simulink model "AUV_ControlsPreliminary"  (R2020b)
(part 12 of 62)

      settings: PortSchema="{\"entries\":[{\"content\":{\"sides\":[{\"content\":{\"connectorIds\":[\"LConn1\"]},\"type\":\"ConnectorPlacement.EquallySpacedRectSide\",\"uuid\":\"a971723f-ea37-4e9b-910b-501b94fb0ba2\"},{\"content\":{\"connectorIds\":[\"RConn1\"],\"side\":\"RIGHT\"},\"type\":\"ConnectorPlacement.EquallySpacedRectSide\",\"uuid\":\"e50175c1-005c-4b0b-bced-b882197eaab2\"},{\"content\":{\"connectorIds\":[\"LConn2\"],\"side\":\"TOP\"},\"type\":\"ConnectorPlacement.EquallySpacedRectSide\",\"uuid\":\"2a04a964-d53e-47ee-8c79-d53dd599bafe\"},{\"content\":{\"connectorIds\":[\"RConn2\"],\"side\":\"BOTTOM\"},\"type\":\"ConnectorPlacement.EquallySpacedRectSide\",\"uuid\":\"a0066dd6-a193-491c-afbe-bac00dfc3505\"}]},\"type\":\"ConnectorPlacement.EquallySpacedConnector\",\"uuid\":\"c80211c6-bb24-481b-97ca-2752015f3b18\"}],\"packageUris\":[\"http://schema.mathworks.com/mf0/Connector/19700101\"],\"version\":\"1.0\"}"
  Tile63 : Subsystem  mask(Square Tile){side=side, thickness=thick, color=color1, opacity=opacity}
      mask prompts: side "Side (m) :"; thickness "Thickness (m) :"; color "Color [RGB] :"; opacity "Opacity (0...1) :"
      mask help: This block creates a flat, single, square tile element. The square tile body is mass-less, so it will not have an effect on the dynamic simulation. This square tile element can be used as a graphic reference by itself, or as part of a composite graphic reference made of an array of interconnected tiles. The square tile is aligned with the XY plane, and the block provides frame connector ports to the middle points on each of the four sides of the body of the square - right (+X), left (-X), top (+Y) and bottom (-Y). All dimensions are in meters.
      settings: PortSchema="{\"entries\":[{\"content\":{\"sides\":[{\"content\":{\"connectorIds\":[\"LConn1\"]},\"type\":\"ConnectorPlacement.EquallySpacedRectSide\",\"uuid\":\"a971723f-ea37-4e9b-910b-501b94fb0ba2\"},{\"content\":{\"connectorIds\":[\"RConn1\"],\"side\":\"RIGHT\"},\"type\":\"ConnectorPlacement.EquallySpacedRectSide\",\"uuid\":\"e50175c1-005c-4b0b-bced-b882197eaab2\"},{\"content\":{\"connectorIds\":[\"LConn2\"],\"side\":\"TOP\"},\"type\":\"ConnectorPlacement.EquallySpacedRectSide\",\"uuid\":\"2a04a964-d53e-47ee-8c79-d53dd599bafe\"},{\"content\":{\"connectorIds\":[\"RConn2\"],\"side\":\"BOTTOM\"},\"type\":\"ConnectorPlacement.EquallySpacedRectSide\",\"uuid\":\"a0066dd6-a193-491c-afbe-bac00dfc3505\"}]},\"type\":\"ConnectorPlacement.EquallySpacedConnector\",\"uuid\":\"c80211c6-bb24-481b-97ca-2752015f3b18\"}],\"packageUris\":[\"http://schema.mathworks.com/mf0/Connector/19700101\"],\"version\":\"1.0\"}"
  Tile64 : Subsystem  mask(Square Tile){side=side, thickness=thick, color=color2, opacity=opacity}
      mask prompts: side "Side (m) :"; thickness "Thickness (m) :"; color "Color [RGB] :"; opacity "Opacity (0...1) :"
      mask help: This block creates a flat, single, square tile element. The square tile body is mass-less, so it will not have an effect on the dynamic simulation. This square tile element can be used as a graphic reference by itself, or as part of a composite graphic reference made of an array of interconnected tiles. The square tile is aligned with the XY plane, and the block provides frame connector ports to the middle points on each of the four sides of the body of the square - right (+X), left (-X), top (+Y) and bottom (-Y). All dimensions are in meters.
      settings: PortSchema="{\"entries\":[{\"content\":{\"sides\":[{\"content\":{\"connectorIds\":[\"LConn1\"]},\"type\":\"ConnectorPlacement.EquallySpacedRectSide\",\"uuid\":\"a971723f-ea37-4e9b-910b-501b94fb0ba2\"},{\"content\":{\"connectorIds\":[\"RConn1\"],\"side\":\"RIGHT\"},\"type\":\"ConnectorPlacement.EquallySpacedRectSide\",\"uuid\":\"e50175c1-005c-4b0b-bced-b882197eaab2\"},{\"content\":{\"connectorIds\":[\"LConn2\"],\"side\":\"TOP\"},\"type\":\"ConnectorPlacement.EquallySpacedRectSide\",\"uuid\":\"2a04a964-d53e-47ee-8c79-d53dd599bafe\"},{\"content\":{\"connectorIds\":[\"RConn2\"],\"side\":\"BOTTOM\"},\"type\":\"ConnectorPlacement.EquallySpacedRectSide\",\"uuid\":\"a0066dd6-a193-491c-afbe-bac00dfc3505\"}]},\"type\":\"ConnectorPlacement.EquallySpacedConnector\",\"uuid\":\"c80211c6-bb24-481b-97ca-2752015f3b18\"}],\"packageUris\":[\"http://schema.mathworks.com/mf0/Connector/19700101\"],\"version\":\"1.0\"}"
  Tile65 : Subsystem  mask(Square Tile){side=side, thickness=thick, color=color1, opacity=opacity}
      mask prompts: side "Side (m) :"; thickness "Thickness (m) :"; color "Color [RGB] :"; opacity "Opacity (0...1) :"
      mask help: This block creates a flat, single, square tile element. The square tile body is mass-less, so it will not have an effect on the dynamic simulation. This square tile element can be used as a graphic reference by itself, or as part of a composite graphic reference made of an array of interconnected tiles. The square tile is aligned with the XY plane, and the block provides frame connector ports to the middle points on each of the four sides of the body of the square - right (+X), left (-X), top (+Y) and bottom (-Y). All dimensions are in meters.
      settings: PortSchema="{\"entries\":[{\"content\":{\"sides\":[{\"content\":{\"connectorIds\":[\"LConn1\"]},\"type\":\"ConnectorPlacement.EquallySpacedRectSide\",\"uuid\":\"a971723f-ea37-4e9b-910b-501b94fb0ba2\"},{\"content\":{\"connectorIds\":[\"RConn1\"],\"side\":\"RIGHT\"},\"type\":\"ConnectorPlacement.EquallySpacedRectSide\",\"uuid\":\"e50175c1-005c-4b0b-bced-b882197eaab2\"},{\"content\":{\"connectorIds\":[\"LConn2\"],\"side\":\"TOP\"},\"type\":\"ConnectorPlacement.EquallySpacedRectSide\",\"uuid\":\"2a04a964-d53e-47ee-8c79-d53dd599bafe\"},{\"content\":{\"connectorIds\":[\"RConn2\"],\"side\":\"BOTTOM\"},\"type\":\"ConnectorPlacement.EquallySpacedRectSide\",\"uuid\":\"a0066dd6-a193-491c-afbe-bac00dfc3505\"}]},\"type\":\"ConnectorPlacement.EquallySpacedConnector\",\"uuid\":\"c80211c6-bb24-481b-97ca-2752015f3b18\"}],\"packageUris\":[\"http://schema.mathworks.com/mf0/Connector/19700101\"],\"version\":\"1.0\"}"
  Tile66 : Subsystem  mask(Square Tile){side=side, thickness=thick, color=color2, opacity=opacity}
      mask prompts: side "Side (m) :"; thickness "Thickness (m) :"; color "Color [RGB] :"; opacity "Opacity (0...1) :"
      mask help: This block creates a flat, single, square tile element. The square tile body is mass-less, so it will not have an effect on the dynamic simulation. This square tile element can be used as a graphic reference by itself, or as part of a composite graphic reference made of an array of interconnected tiles. The square tile is aligned with the XY plane, and the block provides frame connector ports to the middle points on each of the four sides of the body of the square - right (+X), left (-X), top (+Y) and bottom (-Y). All dimensions are in meters.
      settings: PortSchema="{\"entries\":[{\"content\":{\"sides\":[{\"content\":{\"connectorIds\":[\"LConn1\"]},\"type\":\"ConnectorPlacement.EquallySpacedRectSide\",\"uuid\":\"a971723f-ea37-4e9b-910b-501b94fb0ba2\"},{\"content\":{\"connectorIds\":[\"RConn1\"],\"side\":\"RIGHT\"},\"type\":\"ConnectorPlacement.EquallySpacedRectSide\",\"uuid\":\"e50175c1-005c-4b0b-bced-b882197eaab2\"},{\"content\":{\"connectorIds\":[\"LConn2\"],\"side\":\"TOP\"},\"type\":\"ConnectorPlacement.EquallySpacedRectSide\",\"uuid\":\"2a04a964-d53e-47ee-8c79-d53dd599bafe\"},{\"content\":{\"connectorIds\":[\"RConn2\"],\"side\":\"BOTTOM\"},\"type\":\"ConnectorPlacement.EquallySpacedRectSide\",\"uuid\":\"a0066dd6-a193-491c-afbe-bac00dfc3505\"}]},\"type\":\"ConnectorPlacement.EquallySpacedConnector\",\"uuid\":\"c80211c6-bb24-481b-97ca-2752015f3b18\"}],\"packageUris\":[\"http://schema.mathworks.com/mf0/Connector/19700101\"],\"version\":\"1.0\"}"
  Tile67 : Subsystem  mask(Square Tile){side=side, thickness=thick, color=color1, opacity=opacity}
      mask prompts: side "Side (m) :"; thickness "Thickness (m) :"; color "Color [RGB] :"; opacity "Opacity (0...1) :"
      mask help: This block creates a flat, single, square tile element. The square tile body is mass-less, so it will not have an effect on the dynamic simulation. This square tile element can be used as a graphic reference by itself, or as part of a composite graphic reference made of an array of interconnected tiles. The square tile is aligned with the XY plane, and the block provides frame connector ports to the middle points on each of the four sides of the body of the square - right (+X), left (-X), top (+Y) and bottom (-Y). All dimensions are in meters.
      settings: PortSchema="{\"entries\":[{\"content\":{\"sides\":[{\"content\":{\"connectorIds\":[\"LConn1\"]},\"type\":\"ConnectorPlacement.EquallySpacedRectSide\",\"uuid\":\"a971723f-ea37-4e9b-910b-501b94fb0ba2\"},{\"content\":{\"connectorIds\":[\"RConn1\"],\"side\":\"RIGHT\"},\"type\":\"ConnectorPlacement.EquallySpacedRectSide\",\"uuid\":\"e50175c1-005c-4b0b-bced-b882197eaab2\"},{\"content\":{\"connectorIds\":[\"LConn2\"],\"side\":\"TOP\"},\"type\":\"ConnectorPlacement.EquallySpacedRectSide\",\"uuid\":\"2a04a964-d53e-47ee-8c79-d53dd599bafe\"},{\"content\":{\"connectorIds\":[\"RConn2\"],\"side\":\"BOTTOM\"},\"type\":\"ConnectorPlacement.EquallySpacedRectSide\",\"uuid\":\"a0066dd6-a193-491c-afbe-bac00dfc3505\"}]},\"type\":\"ConnectorPlacement.EquallySpacedConnector\",\"uuid\":\"c80211c6-bb24-481b-97ca-2752015f3b18\"}],\"packageUris\":[\"http://schema.mathworks.com/mf0/Connector/19700101\"],\"version\":\"1.0\"}"
  Tile68 : Subsystem  mask(Square Tile){side=side, thickness=thick, color=color2, opacity=opacity}
      mask prompts: side "Side (m) :"; thickness "Thickness (m) :"; color "Color [RGB] :"; opacity "Opacity (0...1) :"
      mask help: This block creates a flat, single, square tile element. The square tile body is mass-less, so it will not have an effect on the dynamic simulation. This square tile element can be used as a graphic reference by itself, or as part of a composite graphic reference made of an array of interconnected tiles. The square tile is aligned with the XY plane, and the block provides frame connector ports to the middle points on each of the four sides of the body of the square - right (+X), left (-X), top (+Y) and bottom (-Y). All dimensions are in meters.
      settings: PortSchema="{\"entries\":[{\"content\":{\"sides\":[{\"content\":{\"connectorIds\":[\"LConn1\"]},\"type\":\"ConnectorPlacement.EquallySpacedRectSide\",\"uuid\":\"a971723f-ea37-4e9b-910b-501b94fb0ba2\"},{\"content\":{\"connectorIds\":[\"RConn1\"],\"side\":\"RIGHT\"},\"type\":\"ConnectorPlacement.EquallySpacedRectSide\",\"uuid\":\"e50175c1-005c-4b0b-bced-b882197eaab2\"},{\"content\":{\"connectorIds\":[\"LConn2\"],\"side\":\"TOP\"},\"type\":\"ConnectorPlacement.EquallySpacedRectSide\",\"uuid\":\"2a04a964-d53e-47ee-8c79-d53dd599bafe\"},{\"content\":{\"connectorIds\":[\"RConn2\"],\"side\":\"BOTTOM\"},\"type\":\"ConnectorPlacement.EquallySpacedRectSide\",\"uuid\":\"a0066dd6-a193-491c-afbe-bac00dfc3505\"}]},\"type\":\"ConnectorPlacement.EquallySpacedConnector\",\"uuid\":\"c80211c6-bb24-481b-97ca-2752015f3b18\"}],\"packageUris\":[\"http://schema.mathworks.com/mf0/Connector/19700101\"],\"version\":\"1.0\"}"
  Tile69 : Subsystem  mask(Square Tile){side=side, thickness=thick, color=color1, opacity=opacity}
      mask prompts: side "Side (m) :"; thickness "Thickness (m) :"; color "Color [RGB] :"; opacity "Opacity (0...1) :"
      mask help: This block creates a flat, single, square tile element. The square tile body is mass-less, so it will not have an effect on the dynamic simulation. This square tile element can be used as a graphic reference by itself, or as part of a composite graphic reference made of an array of interconnected tiles. The square tile is aligned with the XY plane, and the block provides frame connector ports to the middle points on each of the four sides of the body of the square - right (+X), left (-X), top (+Y) and bottom (-Y). All dimensions are in meters.
      settings: PortSchema="{\"entries\":[{\"content\":{\"sides\":[{\"content\":{\"connectorIds\":[\"LConn1\"]},\"type\":\"ConnectorPlacement.EquallySpacedRectSide\",\"uuid\":\"a971723f-ea37-4e9b-910b-501b94fb0ba2\"},{\"content\":{\"connectorIds\":[\"RConn1\"],\"side\":\"RIGHT\"},\"type\":\"ConnectorPlacement.EquallySpacedRectSide\",\"uuid\":\"e50175c1-005c-4b0b-bced-b882197eaab2\"},{\"content\":{\"connectorIds\":[\"LConn2\"],\"side\":\"TOP\"},\"type\":\"ConnectorPlacement.EquallySpacedRectSide\",\"uuid\":\"2a04a964-d53e-47ee-8c79-d53dd599bafe\"},{\"content\":{\"connectorIds\":[\"RConn2\"],\"side\":\"BOTTOM\"},\"type\":\"ConnectorPlacement.EquallySpacedRectSide\",\"uuid\":\"a0066dd6-a193-491c-afbe-bac00dfc3505\"}]},\"type\":\"ConnectorPlacement.EquallySpacedConnector\",\"uuid\":\"c80211c6-bb24-481b-97ca-2752015f3b18\"}],\"packageUris\":[\"http://schema.mathworks.com/mf0/Connector/19700101\"],\"version\":\"1.0\"}"
  Tile7 : Subsystem  mask(Square Tile){side=side, thickness=thick, color=color1, opacity=opacity}
      mask prompts: side "Side (m) :"; thickness "Thickness (m) :"; color "Color [RGB] :"; opacity "Opacity (0...1) :"
      mask help: This block creates a flat, single, square tile element. The square tile body is mass-less, so it will not have an effect on the dynamic simulation. This square tile element can be used as a graphic reference by itself, or as part of a composite graphic reference made of an array of interconnected tiles. The square tile is aligned with the XY plane, and the block provides frame connector ports to the middle points on each of the four sides of the body of the square - right (+X), left (-X), top (+Y) and bottom (-Y). All dimensions are in meters.
      settings: PortSchema="{\"entries\":[{\"content\":{\"sides\":[{\"content\":{\"connectorIds\":[\"LConn1\"]},\"type\":\"ConnectorPlacement.EquallySpacedRectSide\",\"uuid\":\"a971723f-ea37-4e9b-910b-501b94fb0ba2\"},{\"content\":{\"connectorIds\":[\"RConn1\"],\"side\":\"RIGHT\"},\"type\":\"ConnectorPlacement.EquallySpacedRectSide\",\"uuid\":\"e50175c1-005c-4b0b-bced-b882197eaab2\"},{\"content\":{\"connectorIds\":[\"LConn2\"],\"side\":\"TOP\"},\"type\":\"ConnectorPlacement.EquallySpacedRectSide\",\"uuid\":\"2a04a964-d53e-47ee-8c79-d53dd599bafe\"},{\"content\":{\"connectorIds\":[\"RConn2\"],\"side\":\"BOTTOM\"},\"type\":\"ConnectorPlacement.EquallySpacedRectSide\",\"uuid\":\"a0066dd6-a193-491c-afbe-bac00dfc3505\"}]},\"type\":\"ConnectorPlacement.EquallySpacedConnector\",\"uuid\":\"c80211c6-bb24-481b-97ca-2752015f3b18\"}],\"packageUris\":[\"http://schema.mathworks.com/mf0/Connector/19700101\"],\"version\":\"1.0\"}"
  Tile70 : Subsystem  mask(Square Tile){side=side, thickness=thick, color=color1, opacity=opacity}
      mask prompts: side "Side (m) :"; thickness "Thickness (m) :"; color "Color [RGB] :"; opacity "Opacity (0...1) :"
      mask help: This block creates a flat, single, square tile element. The square tile body is mass-less, so it will not have an effect on the dynamic simulation. This square tile element can be used as a graphic reference by itself, or as part of a composite graphic reference made of an array of interconnected tiles. The square tile is aligned with the XY plane, and the block provides frame connector ports to the middle points on each of the four sides of the body of the square - right (+X), left (-X), top (+Y) and bottom (-Y). All dimensions are in meters.
      settings: PortSchema="{\"entries\":[{\"content\":{\"sides\":[{\"content\":{\"connectorIds\":[\"LConn1\"]},\"type\":\"ConnectorPlacement.EquallySpacedRectSide\",\"uuid\":\"a971723f-ea37-4e9b-910b-501b94fb0ba2\"},{\"content\":{\"connectorIds\":[\"RConn1\"],\"side\":\"RIGHT\"},\"type\":\"ConnectorPlacement.EquallySpacedRectSide\",\"uuid\":\"e50175c1-005c-4b0b-bced-b882197eaab2\"},{\"content\":{\"connectorIds\":[\"LConn2\"],\"side\":\"TOP\"},\"type\":\"ConnectorPlacement.EquallySpacedRectSide\",\"uuid\":\"2a04a964-d53e-47ee-8c79-d53dd599bafe\"},{\"content\":{\"connectorIds\":[\"RConn2\"],\"side\":\"BOTTOM\"},\"type\":\"ConnectorPlacement.EquallySpacedRectSide\",\"uuid\":\"a0066dd6-a193-491c-afbe-bac00dfc3505\"}]},\"type\":\"ConnectorPlacement.EquallySpacedConnector\",\"uuid\":\"c80211c6-bb24-481b-97ca-2752015f3b18\"}],\"packageUris\":[\"http://schema.mathworks.com/mf0/Connector/19700101\"],\"version\":\"1.0\"}"
  Tile71 : Subsystem  mask(Square Tile){side=side, thickness=thick, color=color1, opacity=opacity}
      mask prompts: side "Side (m) :"; thickness "Thickness (m) :"; color "Color [RGB] :"; opacity "Opacity (0...1) :"
      mask help: This block creates a flat, single, square tile element. The square tile body is mass-less, so it will not have an effect on the dynamic simulation. This square tile element can be used as a graphic reference by itself, or as part of a composite graphic reference made of an array of interconnected tiles. The square tile is aligned with the XY plane, and the block provides frame connector ports to the middle points on each of the four sides of the body of the square - right (+X), left (-X), top (+Y) and bottom (-Y). All dimensions are in meters.
      settings: PortSchema="{\"entries\":[{\"content\":{\"sides\":[{\"content\":{\"connectorIds\":[\"LConn1\"]},\"type\":\"ConnectorPlacement.EquallySpacedRectSide\",\"uuid\":\"a971723f-ea37-4e9b-910b-501b94fb0ba2\"},{\"content\":{\"connectorIds\":[\"RConn1\"],\"side\":\"RIGHT\"},\"type\":\"ConnectorPlacement.EquallySpacedRectSide\",\"uuid\":\"e50175c1-005c-4b0b-bced-b882197eaab2\"},{\"content\":{\"connectorIds\":[\"LConn2\"],\"side\":\"TOP\"},\"type\":\"ConnectorPlacement.EquallySpacedRectSide\",\"uuid\":\"2a04a964-d53e-47ee-8c79-d53dd599bafe\"},{\"content\":{\"connectorIds\":[\"RConn2\"],\"side\":\"BOTTOM\"},\"type\":\"ConnectorPlacement.EquallySpacedRectSide\",\"uuid\":\"a0066dd6-a193-491c-afbe-bac00dfc3505\"}]},\"type\":\"ConnectorPlacement.EquallySpacedConnector\",\"uuid\":\"c80211c6-bb24-481b-97ca-2752015f3b18\"}],\"packageUris\":[\"http://schema.mathworks.com/mf0/Connector/19700101\"],\"version\":\"1.0\"}"
  Tile72 : Subsystem  mask(Square Tile){side=side, thickness=thick, color=color2, opacity=opacity}
      mask prompts: side "Side (m) :"; thickness "Thickness (m) :"; color "Color [RGB] :"; opacity "Opacity (0...1) :"
      mask help: This block creates a flat, single, square tile element. The square tile body is mass-less, so it will not have an effect on the dynamic simulation. This square tile element can be used as a graphic reference by itself, or as part of a composite graphic reference made of an array of interconnected tiles. The square tile is aligned with the XY plane, and the block provides frame connector ports to the middle points on each of the four sides of the body of the square - right (+X), left (-X), top (+Y) and bottom (-Y). All dimensions are in meters.
      settings: PortSchema="{\"entries\":[{\"content\":{\"sides\":[{\"content\":{\"connectorIds\":[\"LConn1\"]},\"type\":\"ConnectorPlacement.EquallySpacedRectSide\",\"uuid\":\"a971723f-ea37-4e9b-910b-501b94fb0ba2\"},{\"content\":{\"connectorIds\":[\"RConn1\"],\"side\":\"RIGHT\"},\"type\":\"ConnectorPlacement.EquallySpacedRectSide\",\"uuid\":\"e50175c1-005c-4b0b-bced-b882197eaab2\"},{\"content\":{\"connectorIds\":[\"LConn2\"],\"side\":\"TOP\"},\"type\":\"ConnectorPlacement.EquallySpacedRectSide\",\"uuid\":\"2a04a964-d53e-47ee-8c79-d53dd599bafe\"},{\"content\":{\"connectorIds\":[\"RConn2\"],\"side\":\"BOTTOM\"},\"type\":\"ConnectorPlacement.EquallySpacedRectSide\",\"uuid\":\"a0066dd6-a193-491c-afbe-bac00dfc3505\"}]},\"type\":\"ConnectorPlacement.EquallySpacedConnector\",\"uuid\":\"c80211c6-bb24-481b-97ca-2752015f3b18\"}],\"packageUris\":[\"http://schema.mathworks.com/mf0/Connector/19700101\"],\"version\":\"1.0\"}"
  Tile73 : Subsystem  mask(Square Tile){side=side, thickness=thick, color=color2, opacity=opacity}
      mask prompts: side "Side (m) :"; thickness "Thickness (m) :"; color "Color [RGB] :"; opacity "Opacity (0...1) :"
      mask help: This block creates a flat, single, square tile element. The square tile body is mass-less, so it will not have an effect on the dynamic simulation. This square tile element can be used as a graphic reference by itself, or as part of a composite graphic reference made of an array of interconnected tiles. The square tile is aligned with the XY plane, and the block provides frame connector ports to the middle points on each of the four sides of the body of the square - right (+X), left (-X), top (+Y) and bottom (-Y). All dimensions are in meters.
      settings: PortSchema="{\"entries\":[{\"content\":{\"sides\":[{\"content\":{\"connectorIds\":[\"LConn1\"]},\"type\":\"ConnectorPlacement.EquallySpacedRectSide\",\"uuid\":\"a971723f-ea37-4e9b-910b-501b94fb0ba2\"},{\"content\":{\"connectorIds\":[\"RConn1\"],\"side\":\"RIGHT\"},\"type\":\"ConnectorPlacement.EquallySpacedRectSide\",\"uuid\":\"e50175c1-005c-4b0b-bced-b882197eaab2\"},{\"content\":{\"connectorIds\":[\"LConn2\"],\"side\":\"TOP\"},\"type\":\"ConnectorPlacement.EquallySpacedRectSide\",\"uuid\":\"2a04a964-d53e-47ee-8c79-d53dd599bafe\"},{\"content\":{\"connectorIds\":[\"RConn2\"],\"side\":\"BOTTOM\"},\"type\":\"ConnectorPlacement.EquallySpacedRectSide\",\"uuid\":\"a0066dd6-a193-491c-afbe-bac00dfc3505\"}]},\"type\":\"ConnectorPlacement.EquallySpacedConnector\",\"uuid\":\"c80211c6-bb24-481b-97ca-2752015f3b18\"}],\"packageUris\":[\"http://schema.mathworks.com/mf0/Connector/19700101\"],\"version\":\"1.0\"}"
  Tile74 : Subsystem  mask(Square Tile){side=side, thickness=thick, color=color2, opacity=opacity}
      mask prompts: side "Side (m) :"; thickness "Thickness (m) :"; color "Color [RGB] :"; opacity "Opacity (0...1) :"
      mask help: This block creates a flat, single, square tile element. The square tile body is mass-less, so it will not have an effect on the dynamic simulation. This square tile element can be used as a graphic reference by itself, or as part of a composite graphic reference made of an array of interconnected tiles. The square tile is aligned with the XY plane, and the block provides frame connector ports to the middle points on each of the four sides of the body of the square - right (+X), left (-X), top (+Y) and bottom (-Y). All dimensions are in meters.
      settings: PortSchema="{\"entries\":[{\"content\":{\"sides\":[{\"content\":{\"connectorIds\":[\"LConn1\"]},\"type\":\"ConnectorPlacement.EquallySpacedRectSide\",\"uuid\":\"a971723f-ea37-4e9b-910b-501b94fb0ba2\"},{\"content\":{\"connectorIds\":[\"RConn1\"],\"side\":\"RIGHT\"},\"type\":\"ConnectorPlacement.EquallySpacedRectSide\",\"uuid\":\"e50175c1-005c-4b0b-bced-b882197eaab2\"},{\"content\":{\"connectorIds\":[\"LConn2\"],\"side\":\"TOP\"},\"type\":\"ConnectorPlacement.EquallySpacedRectSide\",\"uuid\":\"2a04a964-d53e-47ee-8c79-d53dd599bafe\"},{\"content\":{\"connectorIds\":[\"RConn2\"],\"side\":\"BOTTOM\"},\"type\":\"ConnectorPlacement.EquallySpacedRectSide\",\"uuid\":\"a0066dd6-a193-491c-afbe-bac00dfc3505\"}]},\"type\":\"ConnectorPlacement.EquallySpacedConnector\",\"uuid\":\"c80211c6-bb24-481b-97ca-2752015f3b18\"}],\"packageUris\":[\"http://schema.mathworks.com/mf0/Connector/19700101\"],\"version\":\"1.0\"}"
  Tile75 : Subsystem  mask(Square Tile){side=side, thickness=thick, color=color1, opacity=opacity}
      mask prompts: side "Side (m) :"; thickness "Thickness (m) :"; color "Color [RGB] :"; opacity "Opacity (0...1) :"
      mask help: This block creates a flat, single, square tile element. The square tile body is mass-less, so it will not have an effect on the dynamic simulation. This square tile element can be used as a graphic reference by itself, or as part of a composite graphic reference made of an array of interconnected tiles. The square tile is aligned with the XY plane, and the block provides frame connector ports to the middle points on each of the four sides of the body of the square - right (+X), left (-X), top (+Y) and bottom (-Y). All dimensions are in meters.
      settings: PortSchema="{\"entries\":[{\"content\":{\"sides\":[{\"content\":{\"connectorIds\":[\"LConn1\"]},\"type\":\"ConnectorPlacement.EquallySpacedRectSide\",\"uuid\":\"a971723f-ea37-4e9b-910b-501b94fb0ba2\"},{\"content\":{\"connectorIds\":[\"RConn1\"],\"side\":\"RIGHT\"},\"type\":\"ConnectorPlacement.EquallySpacedRectSide\",\"uuid\":\"e50175c1-005c-4b0b-bced-b882197eaab2\"},{\"content\":{\"connectorIds\":[\"LConn2\"],\"side\":\"TOP\"},\"type\":\"ConnectorPlacement.EquallySpacedRectSide\",\"uuid\":\"2a04a964-d53e-47ee-8c79-d53dd599bafe\"},{\"content\":{\"connectorIds\":[\"RConn2\"],\"side\":\"BOTTOM\"},\"type\":\"ConnectorPlacement.EquallySpacedRectSide\",\"uuid\":\"a0066dd6-a193-491c-afbe-bac00dfc3505\"}]},\"type\":\"ConnectorPlacement.EquallySpacedConnector\",\"uuid\":\"c80211c6-bb24-481b-97ca-2752015f3b18\"}],\"packageUris\":[\"http://schema.mathworks.com/mf0/Connector/19700101\"],\"version\":\"1.0\"}"
  Tile76 : Subsystem  mask(Square Tile){side=side, thickness=thick, color=color2, opacity=opacity}
      mask prompts: side "Side (m) :"; thickness "Thickness (m) :"; color "Color [RGB] :"; opacity "Opacity (0...1) :"
      mask help: This block creates a flat, single, square tile element. The square tile body is mass-less, so it will not have an effect on the dynamic simulation. This square tile element can be used as a graphic reference by itself, or as part of a composite graphic reference made of an array of interconnected tiles. The square tile is aligned with the XY plane, and the block provides frame connector ports to the middle points on each of the four sides of the body of the square - right (+X), left (-X), top (+Y) and bottom (-Y). All dimensions are in meters.
      settings: PortSchema="{\"entries\":[{\"content\":{\"sides\":[{\"content\":{\"connectorIds\":[\"LConn1\"]},\"type\":\"ConnectorPlacement.EquallySpacedRectSide\",\"uuid\":\"a971723f-ea37-4e9b-910b-501b94fb0ba2\"},{\"content\":{\"connectorIds\":[\"RConn1\"],\"side\":\"RIGHT\"},\"type\":\"ConnectorPlacement.EquallySpacedRectSide\",\"uuid\":\"e50175c1-005c-4b0b-bced-b882197eaab2\"},{\"content\":{\"connectorIds\":[\"LConn2\"],\"side\":\"TOP\"},\"type\":\"ConnectorPlacement.EquallySpacedRectSide\",\"uuid\":\"2a04a964-d53e-47ee-8c79-d53dd599bafe\"},{\"content\":{\"connectorIds\":[\"RConn2\"],\"side\":\"BOTTOM\"},\"type\":\"ConnectorPlacement.EquallySpacedRectSide\",\"uuid\":\"a0066dd6-a193-491c-afbe-bac00dfc3505\"}]},\"type\":\"ConnectorPlacement.EquallySpacedConnector\",\"uuid\":\"c80211c6-bb24-481b-97ca-2752015f3b18\"}],\"packageUris\":[\"http://schema.mathworks.com/mf0/Connector/19700101\"],\"version\":\"1.0\"}"
  Tile77 : Subsystem  mask(Square Tile){side=side, thickness=thick, color=color1, opacity=opacity}
      mask prompts: side "Side (m) :"; thickness "Thickness (m) :"; color "Color [RGB] :"; opacity "Opacity (0...1) :"
      mask help: This block creates a flat, single, square tile element. The square tile body is mass-less, so it will not have an effect on the dynamic simulation. This square tile element can be used as a graphic reference by itself, or as part of a composite graphic reference made of an array of interconnected tiles. The square tile is aligned with the XY plane, and the block provides frame connector ports to the middle points on each of the four sides of the body of the square - right (+X), left (-X), top (+Y) and bottom (-Y). All dimensions are in meters.
      settings: PortSchema="{\"entries\":[{\"content\":{\"sides\":[{\"content\":{\"connectorIds\":[\"LConn1\"]},\"type\":\"ConnectorPlacement.EquallySpacedRectSide\",\"uuid\":\"a971723f-ea37-4e9b-910b-501b94fb0ba2\"},{\"content\":{\"connectorIds\":[\"RConn1\"],\"side\":\"RIGHT\"},\"type\":\"ConnectorPlacement.EquallySpacedRectSide\",\"uuid\":\"e50175c1-005c-4b0b-bced-b882197eaab2\"},{\"content\":{\"connectorIds\":[\"LConn2\"],\"side\":\"TOP\"},\"type\":\"ConnectorPlacement.EquallySpacedRectSide\",\"uuid\":\"2a04a964-d53e-47ee-8c79-d53dd599bafe\"},{\"content\":{\"connectorIds\":[\"RConn2\"],\"side\":\"BOTTOM\"},\"type\":\"ConnectorPlacement.EquallySpacedRectSide\",\"uuid\":\"a0066dd6-a193-491c-afbe-bac00dfc3505\"}]},\"type\":\"ConnectorPlacement.EquallySpacedConnector\",\"uuid\":\"c80211c6-bb24-481b-97ca-2752015f3b18\"}],\"packageUris\":[\"http://schema.mathworks.com/mf0/Connector/19700101\"],\"version\":\"1.0\"}"
  Tile78 : Subsystem  mask(Square Tile){side=side, thickness=thick, color=color2, opacity=opacity}
      mask prompts: side "Side (m) :"; thickness "Thickness (m) :"; color "Color [RGB] :"; opacity "Opacity (0...1) :"
      mask help: This block creates a flat, single, square tile element. The square tile body is mass-less, so it will not have an effect on the dynamic simulation. This square tile element can be used as a graphic reference by itself, or as part of a composite graphic reference made of an array of interconnected tiles. The square tile is aligned with the XY plane, and the block provides frame connector ports to the middle points on each of the four sides of the body of the square - right (+X), left (-X), top (+Y) and bottom (-Y). All dimensions are in meters.
      settings: PortSchema="{\"entries\":[{\"content\":{\"sides\":[{\"content\":{\"connectorIds\":[\"LConn1\"]},\"type\":\"ConnectorPlacement.EquallySpacedRectSide\",\"uuid\":\"a971723f-ea37-4e9b-910b-501b94fb0ba2\"},{\"content\":{\"connectorIds\":[\"RConn1\"],\"side\":\"RIGHT\"},\"type\":\"ConnectorPlacement.EquallySpacedRectSide\",\"uuid\":\"e50175c1-005c-4b0b-bced-b882197eaab2\"},{\"content\":{\"connectorIds\":[\"LConn2\"],\"side\":\"TOP\"},\"type\":\"ConnectorPlacement.EquallySpacedRectSide\",\"uuid\":\"2a04a964-d53e-47ee-8c79-d53dd599bafe\"},{\"content\":{\"connectorIds\":[\"RConn2\"],\"side\":\"BOTTOM\"},\"type\":\"ConnectorPlacement.EquallySpacedRectSide\",\"uuid\":\"a0066dd6-a193-491c-afbe-bac00dfc3505\"}]},\"type\":\"ConnectorPlacement.EquallySpacedConnector\",\"uuid\":\"c80211c6-bb24-481b-97ca-2752015f3b18\"}],\"packageUris\":[\"http://schema.mathworks.com/mf0/Connector/19700101\"],\"version\":\"1.0\"}"
  Tile79 : Subsystem  mask(Square Tile){side=side, thickness=thick, color=color1, opacity=opacity}
      mask prompts: side "Side (m) :"; thickness "Thickness (m) :"; color "Color [RGB] :"; opacity "Opacity (0...1) :"
      mask help: This block creates a flat, single, square tile element. The square tile body is mass-less, so it will not have an effect on the dynamic simulation. This square tile element can be used as a graphic reference by itself, or as part of a composite graphic reference made of an array of interconnected tiles. The square tile is aligned with the XY plane, and the block provides frame connector ports to the middle points on each of the four sides of the body of the square - right (+X), left (-X), top (+Y) and bottom (-Y). All dimensions are in meters.
      settings: PortSchema="{\"entries\":[{\"content\":{\"sides\":[{\"content\":{\"connectorIds\":[\"LConn1\"]},\"type\":\"ConnectorPlacement.EquallySpacedRectSide\",\"uuid\":\"a971723f-ea37-4e9b-910b-501b94fb0ba2\"},{\"content\":{\"connectorIds\":[\"RConn1\"],\"side\":\"RIGHT\"},\"type\":\"ConnectorPlacement.EquallySpacedRectSide\",\"uuid\":\"e50175c1-005c-4b0b-bced-b882197eaab2\"},{\"content\":{\"connectorIds\":[\"LConn2\"],\"side\":\"TOP\"},\"type\":\"ConnectorPlacement.EquallySpacedRectSide\",\"uuid\":\"2a04a964-d53e-47ee-8c79-d53dd599bafe\"},{\"content\":{\"connectorIds\":[\"RConn2\"],\"side\":\"BOTTOM\"},\"type\":\"ConnectorPlacement.EquallySpacedRectSide\",\"uuid\":\"a0066dd6-a193-491c-afbe-bac00dfc3505\"}]},\"type\":\"ConnectorPlacement.EquallySpacedConnector\",\"uuid\":\"c80211c6-bb24-481b-97ca-2752015f3b18\"}],\"packageUris\":[\"http://schema.mathworks.com/mf0/Connector/19700101\"],\"version\":\"1.0\"}"
  Tile8 : Subsystem  mask(Square Tile){side=side, thickness=thick, color=color2, opacity=opacity}
      mask prompts: side "Side (m) :"; thickness "Thickness (m) :"; color "Color [RGB] :"; opacity "Opacity (0...1) :"
      mask help: This block creates a flat, single, square tile element. The square tile body is mass-less, so it will not have an effect on the dynamic simulation. This square tile element can be used as a graphic reference by itself, or as part of a composite graphic reference made of an array of interconnected tiles. The square tile is aligned with the XY plane, and the block provides frame connector ports to the middle points on each of the four sides of the body of the square - right (+X), left (-X), top (+Y) and bottom (-Y). All dimensions are in meters.
      settings: PortSchema="{\"entries\":[{\"content\":{\"sides\":[{\"content\":{\"connectorIds\":[\"LConn1\"]},\"type\":\"ConnectorPlacement.EquallySpacedRectSide\",\"uuid\":\"a971723f-ea37-4e9b-910b-501b94fb0ba2\"},{\"content\":{\"connectorIds\":[\"RConn1\"],\"side\":\"RIGHT\"},\"type\":\"ConnectorPlacement.EquallySpacedRectSide\",\"uuid\":\"e50175c1-005c-4b0b-bced-b882197eaab2\"},{\"content\":{\"connectorIds\":[\"LConn2\"],\"side\":\"TOP\"},\"type\":\"ConnectorPlacement.EquallySpacedRectSide\",\"uuid\":\"2a04a964-d53e-47ee-8c79-d53dd599bafe\"},{\"content\":{\"connectorIds\":[\"RConn2\"],\"side\":\"BOTTOM\"},\"type\":\"ConnectorPlacement.EquallySpacedRectSide\",\"uuid\":\"a0066dd6-a193-491c-afbe-bac00dfc3505\"}]},\"type\":\"ConnectorPlacement.EquallySpacedConnector\",\"uuid\":\"c80211c6-bb24-481b-97ca-2752015f3b18\"}],\"packageUris\":[\"http://schema.mathworks.com/mf0/Connector/19700101\"],\"version\":\"1.0\"}"
  Tile80 : Subsystem  mask(Square Tile){side=side, thickness=thick, color=color2, opacity=opacity}
      mask prompts: side "Side (m) :"; thickness "Thickness (m) :"; color "Color [RGB] :"; opacity "Opacity (0...1) :"
      mask help: This block creates a flat, single, square tile element. The square tile body is mass-less, so it will not have an effect on the dynamic simulation. This square tile element can be used as a graphic reference by itself, or as part of a composite graphic reference made of an array of interconnected tiles. The square tile is aligned with the XY plane, and the block provides frame connector ports to the middle points on each of the four sides of the body of the square - right (+X), left (-X), top (+Y) and bottom (-Y). All dimensions are in meters.
      settings: PortSchema="{\"entries\":[{\"content\":{\"sides\":[{\"content\":{\"connectorIds\":[\"LConn1\"]},\"type\":\"ConnectorPlacement.EquallySpacedRectSide\",\"uuid\":\"a971723f-ea37-4e9b-910b-501b94fb0ba2\"},{\"content\":{\"connectorIds\":[\"RConn1\"],\"side\":\"RIGHT\"},\"type\":\"ConnectorPlacement.EquallySpacedRectSide\",\"uuid\":\"e50175c1-005c-4b0b-bced-b882197eaab2\"},{\"content\":{\"connectorIds\":[\"LConn2\"],\"side\":\"TOP\"},\"type\":\"ConnectorPlacement.EquallySpacedRectSide\",\"uuid\":\"2a04a964-d53e-47ee-8c79-d53dd599bafe\"},{\"content\":{\"connectorIds\":[\"RConn2\"],\"side\":\"BOTTOM\"},\"type\":\"ConnectorPlacement.EquallySpacedRectSide\",\"uuid\":\"a0066dd6-a193-491c-afbe-bac00dfc3505\"}]},\"type\":\"ConnectorPlacement.EquallySpacedConnector\",\"uuid\":\"c80211c6-bb24-481b-97ca-2752015f3b18\"}],\"packageUris\":[\"http://schema.mathworks.com/mf0/Connector/19700101\"],\"version\":\"1.0\"}"
  Tile81 : Subsystem  mask(Square Tile){side=side, thickness=thick, color=color1, opacity=opacity}
      mask prompts: side "Side (m) :"; thickness "Thickness (m) :"; color "Color [RGB] :"; opacity "Opacity (0...1) :"
      mask help: This block creates a flat, single, square tile element. The square tile body is mass-less, so it will not have an effect on the dynamic simulation. This square tile element can be used as a graphic reference by itself, or as part of a composite graphic reference made of an array of interconnected tiles. The square tile is aligned with the XY plane, and the block provides frame connector ports to the middle points on each of the four sides of the body of the square - right (+X), left (-X), top (+Y) and bottom (-Y). All dimensions are in meters.
      settings: PortSchema="{\"entries\":[{\"content\":{\"sides\":[{\"content\":{\"connectorIds\":[\"LConn1\"]},\"type\":\"ConnectorPlacement.EquallySpacedRectSide\",\"uuid\":\"a971723f-ea37-4e9b-910b-501b94fb0ba2\"},{\"content\":{\"connectorIds\":[\"RConn1\"],\"side\":\"RIGHT\"},\"type\":\"ConnectorPlacement.EquallySpacedRectSide\",\"uuid\":\"e50175c1-005c-4b0b-bced-b882197eaab2\"},{\"content\":{\"connectorIds\":[\"LConn2\"],\"side\":\"TOP\"},\"type\":\"ConnectorPlacement.EquallySpacedRectSide\",\"uuid\":\"2a04a964-d53e-47ee-8c79-d53dd599bafe\"},{\"content\":{\"connectorIds\":[\"RConn2\"],\"side\":\"BOTTOM\"},\"type\":\"ConnectorPlacement.EquallySpacedRectSide\",\"uuid\":\"a0066dd6-a193-491c-afbe-bac00dfc3505\"}]},\"type\":\"ConnectorPlacement.EquallySpacedConnector\",\"uuid\":\"c80211c6-bb24-481b-97ca-2752015f3b18\"}],\"packageUris\":[\"http://schema.mathworks.com/mf0/Connector/19700101\"],\"version\":\"1.0\"}"
  Tile82 : Subsystem  mask(Square Tile){side=side, thickness=thick, color=color2, opacity=opacity}
      mask prompts: side "Side (m) :"; thickness "Thickness (m) :"; color "Color [RGB] :"; opacity "Opacity (0...1) :"
      mask help: This block creates a flat, single, square tile element. The square tile body is mass-less, so it will not have an effect on the dynamic simulation. This square tile element can be used as a graphic reference by itself, or as part of a composite graphic reference made of an array of interconnected tiles. The square tile is aligned with the XY plane, and the block provides frame connector ports to the middle points on each of the four sides of the body of the square - right (+X), left (-X), top (+Y) and bottom (-Y). All dimensions are in meters.
      settings: PortSchema="{\"entries\":[{\"content\":{\"sides\":[{\"content\":{\"connectorIds\":[\"LConn1\"]},\"type\":\"ConnectorPlacement.EquallySpacedRectSide\",\"uuid\":\"a971723f-ea37-4e9b-910b-501b94fb0ba2\"},{\"content\":{\"connectorIds\":[\"RConn1\"],\"side\":\"RIGHT\"},\"type\":\"ConnectorPlacement.EquallySpacedRectSide\",\"uuid\":\"e50175c1-005c-4b0b-bced-b882197eaab2\"},{\"content\":{\"connectorIds\":[\"LConn2\"],\"side\":\"TOP\"},\"type\":\"ConnectorPlacement.EquallySpacedRectSide\",\"uuid\":\"2a04a964-d53e-47ee-8c79-d53dd599bafe\"},{\"content\":{\"connectorIds\":[\"RConn2\"],\"side\":\"BOTTOM\"},\"type\":\"ConnectorPlacement.EquallySpacedRectSide\",\"uuid\":\"a0066dd6-a193-491c-afbe-bac00dfc3505\"}]},\"type\":\"ConnectorPlacement.EquallySpacedConnector\",\"uuid\":\"c80211c6-bb24-481b-97ca-2752015f3b18\"}],\"packageUris\":[\"http://schema.mathworks.com/mf0/Connector/19700101\"],\"version\":\"1.0\"}"
  Tile83 : Subsystem  mask(Square Tile){side=side, thickness=thick, color=color1, opacity=opacity}
      mask prompts: side "Side (m) :"; thickness "Thickness (m) :"; color "Color [RGB] :"; opacity "Opacity (0...1) :"
      mask help: This block creates a flat, single, square tile element. The square tile body is mass-less, so it will not have an effect on the dynamic simulation. This square tile element can be used as a graphic reference by itself, or as part of a composite graphic reference made of an array of interconnected tiles. The square tile is aligned with the XY plane, and the block provides frame connector ports to the middle points on each of the four sides of the body of the square - right (+X), left (-X), top (+Y) and bottom (-Y). All dimensions are in meters.
      settings: PortSchema="{\"entries\":[{\"content\":{\"sides\":[{\"content\":{\"connectorIds\":[\"LConn1\"]},\"type\":\"ConnectorPlacement.EquallySpacedRectSide\",\"uuid\":\"a971723f-ea37-4e9b-910b-501b94fb0ba2\"},{\"content\":{\"connectorIds\":[\"RConn1\"],\"side\":\"RIGHT\"},\"type\":\"ConnectorPlacement.EquallySpacedRectSide\",\"uuid\":\"e50175c1-005c-4b0b-bced-b882197eaab2\"},{\"content\":{\"connectorIds\":[\"LConn2\"],\"side\":\"TOP\"},\"type\":\"ConnectorPlacement.EquallySpacedRectSide\",\"uuid\":\"2a04a964-d53e-47ee-8c79-d53dd599bafe\"},{\"content\":{\"connectorIds\":[\"RConn2\"],\"side\":\"BOTTOM\"},\"type\":\"ConnectorPlacement.EquallySpacedRectSide\",\"uuid\":\"a0066dd6-a193-491c-afbe-bac00dfc3505\"}]},\"type\":\"ConnectorPlacement.EquallySpacedConnector\",\"uuid\":\"c80211c6-bb24-481b-97ca-2752015f3b18\"}],\"packageUris\":[\"http://schema.mathworks.com/mf0/Connector/19700101\"],\"version\":\"1.0\"}"
  Tile84 : Subsystem  mask(Square Tile){side=side, thickness=thick, color=color1, opacity=opacity}
      mask prompts: side "Side (m) :"; thickness "Thickness (m) :"; color "Color [RGB] :"; opacity "Opacity (0...1) :"
      mask help: This block creates a flat, single, square tile element. The square tile body is mass-less, so it will not have an effect on the dynamic simulation. This square tile element can be used as a graphic reference by itself, or as part of a composite graphic reference made of an array of interconnected tiles. The square tile is aligned with the XY plane, and the block provides frame connector ports to the middle points on each of the four sides of the body of the square - right (+X), left (-X), top (+Y) and bottom (-Y). All dimensions are in meters.
      settings: PortSchema="{\"entries\":[{\"content\":{\"sides\":[{\"content\":{\"connectorIds\":[\"LConn1\"]},\"type\":\"ConnectorPlacement.EquallySpacedRectSide\",\"uuid\":\"a971723f-ea37-4e9b-910b-501b94fb0ba2\"},{\"content\":{\"connectorIds\":[\"RConn1\"],\"side\":\"RIGHT\"},\"type\":\"ConnectorPlacement.EquallySpacedRectSide\",\"uuid\":\"e50175c1-005c-4b0b-bced-b882197eaab2\"},{\"content\":{\"connectorIds\":[\"LConn2\"],\"side\":\"TOP\"},\"type\":\"ConnectorPlacement.EquallySpacedRectSide\",\"uuid\":\"2a04a964-d53e-47ee-8c79-d53dd599bafe\"},{\"content\":{\"connectorIds\":[\"RConn2\"],\"side\":\"BOTTOM\"},\"type\":\"ConnectorPlacement.EquallySpacedRectSide\",\"uuid\":\"a0066dd6-a193-491c-afbe-bac00dfc3505\"}]},\"type\":\"ConnectorPlacement.EquallySpacedConnector\",\"uuid\":\"c80211c6-bb24-481b-97ca-2752015f3b18\"}],\"packageUris\":[\"http://schema.mathworks.com/mf0/Connector/19700101\"],\"version\":\"1.0\"}"
  Tile85 : Subsystem  mask(Square Tile){side=side, thickness=thick, color=color2, opacity=opacity}
      mask prompts: side "Side (m) :"; thickness "Thickness (m) :"; color "Color [RGB] :"; opacity "Opacity (0...1) :"
      mask help: This block creates a flat, single, square tile element. The square tile body is mass-less, so it will not have an effect on the dynamic simulation. This square tile element can be used as a graphic reference by itself, or as part of a composite graphic reference made of an array of interconnected tiles. The square tile is aligned with the XY plane, and the block provides frame connector ports to the middle points on each of the four sides of the body of the square - right (+X), left (-X), top (+Y) and bottom (-Y). All dimensions are in meters.
      settings: PortSchema="{\"entries\":[{\"content\":{\"sides\":[{\"content\":{\"connectorIds\":[\"LConn1\"]},\"type\":\"ConnectorPlacement.EquallySpacedRectSide\",\"uuid\":\"a971723f-ea37-4e9b-910b-501b94fb0ba2\"},{\"content\":{\"connectorIds\":[\"RConn1\"],\"side\":\"RIGHT\"},\"type\":\"ConnectorPlacement.EquallySpacedRectSide\",\"uuid\":\"e50175c1-005c-4b0b-bced-b882197eaab2\"},{\"content\":{\"connectorIds\":[\"LConn2\"],\"side\":\"TOP\"},\"type\":\"ConnectorPlacement.EquallySpacedRectSide\",\"uuid\":\"2a04a964-d53e-47ee-8c79-d53dd599bafe\"},{\"content\":{\"connectorIds\":[\"RConn2\"],\"side\":\"BOTTOM\"},\"type\":\"ConnectorPlacement.EquallySpacedRectSide\",\"uuid\":\"a0066dd6-a193-491c-afbe-bac00dfc3505\"}]},\"type\":\"ConnectorPlacement.EquallySpacedConnector\",\"uuid\":\"c80211c6-bb24-481b-97ca-2752015f3b18\"}],\"packageUris\":[\"http://schema.mathworks.com/mf0/Connector/19700101\"],\"version\":\"1.0\"}"
  Tile86 : Subsystem  mask(Square Tile){side=side, thickness=thick, color=color1, opacity=opacity}
      mask prompts: side "Side (m) :"; thickness "Thickness (m) :"; color "Color [RGB] :"; opacity "Opacity (0...1) :"
      mask help: This block creates a flat, single, square tile element. The square tile body is mass-less, so it will not have an effect on the dynamic simulation. This square tile element can be used as a graphic reference by itself, or as part of a composite graphic reference made of an array of interconnected tiles. The square tile is aligned with the XY plane, and the block provides frame connector ports to the middle points on each of the four sides of the body of the square - right (+X), left (-X), top (+Y) and bottom (-Y). All dimensions are in meters.
      settings: PortSchema="{\"entries\":[{\"content\":{\"sides\":[{\"content\":{\"connectorIds\":[\"LConn1\"]},\"type\":\"ConnectorPlacement.EquallySpacedRectSide\",\"uuid\":\"a971723f-ea37-4e9b-910b-501b94fb0ba2\"},{\"content\":{\"connectorIds\":[\"RConn1\"],\"side\":\"RIGHT\"},\"type\":\"ConnectorPlacement.EquallySpacedRectSide\",\"uuid\":\"e50175c1-005c-4b0b-bced-b882197eaab2\"},{\"content\":{\"connectorIds\":[\"LConn2\"],\"side\":\"TOP\"},\"type\":\"ConnectorPlacement.EquallySpacedRectSide\",\"uuid\":\"2a04a964-d53e-47ee-8c79-d53dd599bafe\"},{\"content\":{\"connectorIds\":[\"RConn2\"],\"side\":\"BOTTOM\"},\"type\":\"ConnectorPlacement.EquallySpacedRectSide\",\"uuid\":\"a0066dd6-a193-491c-afbe-bac00dfc3505\"}]},\"type\":\"ConnectorPlacement.EquallySpacedConnector\",\"uuid\":\"c80211c6-bb24-481b-97ca-2752015f3b18\"}],\"packageUris\":[\"http://schema.mathworks.com/mf0/Connector/19700101\"],\"version\":\"1.0\"}"
  Tile87 : Subsystem  mask(Square Tile){side=side, thickness=thick, color=color2, opacity=opacity}
      mask prompts: side "Side (m) :"; thickness "Thickness (m) :"; color "Color [RGB] :"; opacity "Opacity (0...1) :"
      mask help: This block creates a flat, single, square tile element. The square tile body is mass-less, so it will not have an effect on the dynamic simulation. This square tile element can be used as a graphic reference by itself, or as part of a composite graphic reference made of an array of interconnected tiles. The square tile is aligned with the XY plane, and the block provides frame connector ports to the middle points on each of the four sides of the body of the square - right (+X), left (-X), top (+Y) and bottom (-Y). All dimensions are in meters.
      settings: PortSchema="{\"entries\":[{\"content\":{\"sides\":[{\"content\":{\"connectorIds\":[\"LConn1\"]},\"type\":\"ConnectorPlacement.EquallySpacedRectSide\",\"uuid\":\"a971723f-ea37-4e9b-910b-501b94fb0ba2\"},{\"content\":{\"connectorIds\":[\"RConn1\"],\"side\":\"RIGHT\"},\"type\":\"ConnectorPlacement.EquallySpacedRectSide\",\"uuid\":\"e50175c1-005c-4b0b-bced-b882197eaab2\"},{\"content\":{\"connectorIds\":[\"LConn2\"],\"side\":\"TOP\"},\"type\":\"ConnectorPlacement.EquallySpacedRectSide\",\"uuid\":\"2a04a964-d53e-47ee-8c79-d53dd599bafe\"},{\"content\":{\"connectorIds\":[\"RConn2\"],\"side\":\"BOTTOM\"},\"type\":\"ConnectorPlacement.EquallySpacedRectSide\",\"uuid\":\"a0066dd6-a193-491c-afbe-bac00dfc3505\"}]},\"type\":\"ConnectorPlacement.EquallySpacedConnector\",\"uuid\":\"c80211c6-bb24-481b-97ca-2752015f3b18\"}],\"packageUris\":[\"http://schema.mathworks.com/mf0/Connector/19700101\"],\"version\":\"1.0\"}"
  Tile88 : Subsystem  mask(Square Tile){side=side, thickness=thick, color=color1, opacity=opacity}
      mask prompts: side "Side (m) :"; thickness "Thickness (m) :"; color "Color [RGB] :"; opacity "Opacity (0...1) :"
      mask help: This block creates a flat, single, square tile element. The square tile body is mass-less, so it will not have an effect on the dynamic simulation. This square tile element can be used as a graphic reference by itself, or as part of a composite graphic reference made of an array of interconnected tiles. The square tile is aligned with the XY plane, and the block provides frame connector ports to the middle points on each of the four sides of the body of the square - right (+X), left (-X), top (+Y) and bottom (-Y). All dimensions are in meters.
      settings: PortSchema="{\"entries\":[{\"content\":{\"sides\":[{\"content\":{\"connectorIds\":[\"LConn1\"]},\"type\":\"ConnectorPlacement.EquallySpacedRectSide\",\"uuid\":\"a971723f-ea37-4e9b-910b-501b94fb0ba2\"},{\"content\":{\"connectorIds\":[\"RConn1\"],\"side\":\"RIGHT\"},\"type\":\"ConnectorPlacement.EquallySpacedRectSide\",\"uuid\":\"e50175c1-005c-4b0b-bced-b882197eaab2\"},{\"content\":{\"connectorIds\":[\"LConn2\"],\"side\":\"TOP\"},\"type\":\"ConnectorPlacement.EquallySpacedRectSide\",\"uuid\":\"2a04a964-d53e-47ee-8c79-d53dd599bafe\"},{\"content\":{\"connectorIds\":[\"RConn2\"],\"side\":\"BOTTOM\"},\"type\":\"ConnectorPlacement.EquallySpacedRectSide\",\"uuid\":\"a0066dd6-a193-491c-afbe-bac00dfc3505\"}]},\"type\":\"ConnectorPlacement.EquallySpacedConnector\",\"uuid\":\"c80211c6-bb24-481b-97ca-2752015f3b18\"}],\"packageUris\":[\"http://schema.mathworks.com/mf0/Connector/19700101\"],\"version\":\"1.0\"}"
  Tile89 : Subsystem  mask(Square Tile){side=side, thickness=thick, color=color2, opacity=opacity}
      mask prompts: side "Side (m) :"; thickness "Thickness (m) :"; color "Color [RGB] :"; opacity "Opacity (0...1) :"
      mask help: This block creates a flat, single, square tile element. The square tile body is mass-less, so it will not have an effect on the dynamic simulation. This square tile element can be used as a graphic reference by itself, or as part of a composite graphic reference made of an array of interconnected tiles. The square tile is aligned with the XY plane, and the block provides frame connector ports to the middle points on each of the four sides of the body of the square - right (+X), left (-X), top (+Y) and bottom (-Y). All dimensions are in meters.
      settings: PortSchema="{\"entries\":[{\"content\":{\"sides\":[{\"content\":{\"connectorIds\":[\"LConn1\"]},\"type\":\"ConnectorPlacement.EquallySpacedRectSide\",\"uuid\":\"a971723f-ea37-4e9b-910b-501b94fb0ba2\"},{\"content\":{\"connectorIds\":[\"RConn1\"],\"side\":\"RIGHT\"},\"type\":\"ConnectorPlacement.EquallySpacedRectSide\",\"uuid\":\"e50175c1-005c-4b0b-bced-b882197eaab2\"},{\"content\":{\"connectorIds\":[\"LConn2\"],\"side\":\"TOP\"},\"type\":\"ConnectorPlacement.EquallySpacedRectSide\",\"uuid\":\"2a04a964-d53e-47ee-8c79-d53dd599bafe\"},{\"content\":{\"connectorIds\":[\"RConn2\"],\"side\":\"BOTTOM\"},\"type\":\"ConnectorPlacement.EquallySpacedRectSide\",\"uuid\":\"a0066dd6-a193-491c-afbe-bac00dfc3505\"}]},\"type\":\"ConnectorPlacement.EquallySpacedConnector\",\"uuid\":\"c80211c6-bb24-481b-97ca-2752015f3b18\"}],\"packageUris\":[\"http://schema.mathworks.com/mf0/Connector/19700101\"],\"version\":\"1.0\"}"
  Tile9 : Subsystem  mask(Square Tile){side=side, thickness=thick, color=color1, opacity=opacity}
      mask prompts: side "Side (m) :"; thickness "Thickness (m) :"; color "Color [RGB] :"; opacity "Opacity (0...1) :"
      mask help: This block creates a flat, single, square tile element. The square tile body is mass-less, so it will not have an effect on the dynamic simulation. This square tile element can be used as a graphic reference by itself, or as part of a composite graphic reference made of an array of interconnected tiles. The square tile is aligned with the XY plane, and the block provides frame connector ports to the middle points on each of the four sides of the body of the square - right (+X), left (-X), top (+Y) and bottom (-Y). All dimensions are in meters.
      settings: PortSchema="{\"entries\":[{\"content\":{\"sides\":[{\"content\":{\"connectorIds\":[\"LConn1\"]},\"type\":\"ConnectorPlacement.EquallySpacedRectSide\",\"uuid\":\"a971723f-ea37-4e9b-910b-501b94fb0ba2\"},{\"content\":{\"connectorIds\":[\"RConn1\"],\"side\":\"RIGHT\"},\"type\":\"ConnectorPlacement.EquallySpacedRectSide\",\"uuid\":\"e50175c1-005c-4b0b-bced-b882197eaab2\"},{\"content\":{\"connectorIds\":[\"LConn2\"],\"side\":\"TOP\"},\"type\":\"ConnectorPlacement.EquallySpacedRectSide\",\"uuid\":\"2a04a964-d53e-47ee-8c79-d53dd599bafe\"},{\"content\":{\"connectorIds\":[\"RConn2\"],\"side\":\"BOTTOM\"},\"type\":\"ConnectorPlacement.EquallySpacedRectSide\",\"uuid\":\"a0066dd6-a193-491c-afbe-bac00dfc3505\"}]},\"type\":\"ConnectorPlacement.EquallySpacedConnector\",\"uuid\":\"c80211c6-bb24-481b-97ca-2752015f3b18\"}],\"packageUris\":[\"http://schema.mathworks.com/mf0/Connector/19700101\"],\"version\":\"1.0\"}"
  Tile90 : Subsystem  mask(Square Tile){side=side, thickness=thick, color=color1, opacity=opacity}
      mask prompts: side "Side (m) :"; thickness "Thickness (m) :"; color "Color [RGB] :"; opacity "Opacity (0...1) :"
      mask help: This block creates a flat, single, square tile element. The square tile body is mass-less, so it will not have an effect on the dynamic simulation. This square tile element can be used as a graphic reference by itself, or as part of a composite graphic reference made of an array of interconnected tiles. The square tile is aligned with the XY plane, and the block provides frame connector ports to the middle points on each of the four sides of the body of the square - right (+X), left (-X), top (+Y) and bottom (-Y). All dimensions are in meters.
      settings: PortSchema="{\"entries\":[{\"content\":{\"sides\":[{\"content\":{\"connectorIds\":[\"LConn1\"]},\"type\":\"ConnectorPlacement.EquallySpacedRectSide\",\"uuid\":\"a971723f-ea37-4e9b-910b-501b94fb0ba2\"},{\"content\":{\"connectorIds\":[\"RConn1\"],\"side\":\"RIGHT\"},\"type\":\"ConnectorPlacement.EquallySpacedRectSide\",\"uuid\":\"e50175c1-005c-4b0b-bced-b882197eaab2\"},{\"content\":{\"connectorIds\":[\"LConn2\"],\"side\":\"TOP\"},\"type\":\"ConnectorPlacement.EquallySpacedRectSide\",\"uuid\":\"2a04a964-d53e-47ee-8c79-d53dd599bafe\"},{\"content\":{\"connectorIds\":[\"RConn2\"],\"side\":\"BOTTOM\"},\"type\":\"ConnectorPlacement.EquallySpacedRectSide\",\"uuid\":\"a0066dd6-a193-491c-afbe-bac00dfc3505\"}]},\"type\":\"ConnectorPlacement.EquallySpacedConnector\",\"uuid\":\"c80211c6-bb24-481b-97ca-2752015f3b18\"}],\"packageUris\":[\"http://schema.mathworks.com/mf0/Connector/19700101\"],\"version\":\"1.0\"}"
  Tile91 : Subsystem  mask(Square Tile){side=side, thickness=thick, color=color1, opacity=opacity}
      mask prompts: side "Side (m) :"; thickness "Thickness (m) :"; color "Color [RGB] :"; opacity "Opacity (0...1) :"
      mask help: This block creates a flat, single, square tile element. The square tile body is mass-less, so it will not have an effect on the dynamic simulation. This square tile element can be used as a graphic reference by itself, or as part of a composite graphic reference made of an array of interconnected tiles. The square tile is aligned with the XY plane, and the block provides frame connector ports to the middle points on each of the four sides of the body of the square - right (+X), left (-X), top (+Y) and bottom (-Y). All dimensions are in meters.
      settings: PortSchema="{\"entries\":[{\"content\":{\"sides\":[{\"content\":{\"connectorIds\":[\"LConn1\"]},\"type\":\"ConnectorPlacement.EquallySpacedRectSide\",\"uuid\":\"a971723f-ea37-4e9b-910b-501b94fb0ba2\"},{\"content\":{\"connectorIds\":[\"RConn1\"],\"side\":\"RIGHT\"},\"type\":\"ConnectorPlacement.EquallySpacedRectSide\",\"uuid\":\"e50175c1-005c-4b0b-bced-b882197eaab2\"},{\"content\":{\"connectorIds\":[\"LConn2\"],\"side\":\"TOP\"},\"type\":\"ConnectorPlacement.EquallySpacedRectSide\",\"uuid\":\"2a04a964-d53e-47ee-8c79-d53dd599bafe\"},{\"content\":{\"connectorIds\":[\"RConn2\"],\"side\":\"BOTTOM\"},\"type\":\"ConnectorPlacement.EquallySpacedRectSide\",\"uuid\":\"a0066dd6-a193-491c-afbe-bac00dfc3505\"}]},\"type\":\"ConnectorPlacement.EquallySpacedConnector\",\"uuid\":\"c80211c6-bb24-481b-97ca-2752015f3b18\"}],\"packageUris\":[\"http://schema.mathworks.com/mf0/Connector/19700101\"],\"version\":\"1.0\"}"
  Tile92 : Subsystem  mask(Square Tile){side=side, thickness=thick, color=color2, opacity=opacity}
      mask prompts: side "Side (m) :"; thickness "Thickness (m) :"; color "Color [RGB] :"; opacity "Opacity (0...1) :"
      mask help: This block creates a flat, single, square tile element. The square tile body is mass-less, so it will not have an effect on the dynamic simulation. This square tile element can be used as a graphic reference by itself, or as part of a composite graphic reference made of an array of interconnected tiles. The square tile is aligned with the XY plane, and the block provides frame connector ports to the middle points on each of the four sides of the body of the square - right (+X), left (-X), top (+Y) and bottom (-Y). All dimensions are in meters.
      settings: PortSchema="{\"entries\":[{\"content\":{\"sides\":[{\"content\":{\"connectorIds\":[\"LConn1\"]},\"type\":\"ConnectorPlacement.EquallySpacedRectSide\",\"uuid\":\"a971723f-ea37-4e9b-910b-501b94fb0ba2\"},{\"content\":{\"connectorIds\":[\"RConn1\"],\"side\":\"RIGHT\"},\"type\":\"ConnectorPlacement.EquallySpacedRectSide\",\"uuid\":\"e50175c1-005c-4b0b-bced-b882197eaab2\"},{\"content\":{\"connectorIds\":[\"LConn2\"],\"side\":\"TOP\"},\"type\":\"ConnectorPlacement.EquallySpacedRectSide\",\"uuid\":\"2a04a964-d53e-47ee-8c79-d53dd599bafe\"},{\"content\":{\"connectorIds\":[\"RConn2\"],\"side\":\"BOTTOM\"},\"type\":\"ConnectorPlacement.EquallySpacedRectSide\",\"uuid\":\"a0066dd6-a193-491c-afbe-bac00dfc3505\"}]},\"type\":\"ConnectorPlacement.EquallySpacedConnector\",\"uuid\":\"c80211c6-bb24-481b-97ca-2752015f3b18\"}],\"packageUris\":[\"http://schema.mathworks.com/mf0/Connector/19700101\"],\"version\":\"1.0\"}"
  Tile93 : Subsystem  mask(Square Tile){side=side, thickness=thick, color=color2, opacity=opacity}
      mask prompts: side "Side (m) :"; thickness "Thickness (m) :"; color "Color [RGB] :"; opacity "Opacity (0...1) :"
      mask help: This block creates a flat, single, square tile element. The square tile body is mass-less, so it will not have an effect on the dynamic simulation. This square tile element can be used as a graphic reference by itself, or as part of a composite graphic reference made of an array of interconnected tiles. The square tile is aligned with the XY plane, and the block provides frame connector ports to the middle points on each of the four sides of the body of the square - right (+X), left (-X), top (+Y) and bottom (-Y). All dimensions are in meters.
      settings: PortSchema="{\"entries\":[{\"content\":{\"sides\":[{\"content\":{\"connectorIds\":[\"LConn1\"]},\"type\":\"ConnectorPlacement.EquallySpacedRectSide\",\"uuid\":\"a971723f-ea37-4e9b-910b-501b94fb0ba2\"},{\"content\":{\"connectorIds\":[\"RConn1\"],\"side\":\"RIGHT\"},\"type\":\"ConnectorPlacement.EquallySpacedRectSide\",\"uuid\":\"e50175c1-005c-4b0b-bced-b882197eaab2\"},{\"content\":{\"connectorIds\":[\"LConn2\"],\"side\":\"TOP\"},\"type\":\"ConnectorPlacement.EquallySpacedRectSide\",\"uuid\":\"2a04a964-d53e-47ee-8c79-d53dd599bafe\"},{\"content\":{\"connectorIds\":[\"RConn2\"],\"side\":\"BOTTOM\"},\"type\":\"ConnectorPlacement.EquallySpacedRectSide\",\"uuid\":\"a0066dd6-a193-491c-afbe-bac00dfc3505\"}]},\"type\":\"ConnectorPlacement.EquallySpacedConnector\",\"uuid\":\"c80211c6-bb24-481b-97ca-2752015f3b18\"}],\"packageUris\":[\"http://schema.mathworks.com/mf0/Connector/19700101\"],\"version\":\"1.0\"}"
  Tile94 : Subsystem  mask(Square Tile){side=side, thickness=thick, color=color1, opacity=opacity}
      mask prompts: side "Side (m) :"; thickness "Thickness (m) :"; color "Color [RGB] :"; opacity "Opacity (0...1) :"
      mask help: This block creates a flat, single, square tile element. The square tile body is mass-less, so it will not have an effect on the dynamic simulation. This square tile element can be used as a graphic reference by itself, or as part of a composite graphic reference made of an array of interconnected tiles. The square tile is aligned with the XY plane, and the block provides frame connector ports to the middle points on each of the four sides of the body of the square - right (+X), left (-X), top (+Y) and bottom (-Y). All dimensions are in meters.
      settings: PortSchema="{\"entries\":[{\"content\":{\"sides\":[{\"content\":{\"connectorIds\":[\"LConn1\"]},\"type\":\"ConnectorPlacement.EquallySpacedRectSide\",\"uuid\":\"a971723f-ea37-4e9b-910b-501b94fb0ba2\"},{\"content\":{\"connectorIds\":[\"RConn1\"],\"side\":\"RIGHT\"},\"type\":\"ConnectorPlacement.EquallySpacedRectSide\",\"uuid\":\"e50175c1-005c-4b0b-bced-b882197eaab2\"},{\"content\":{\"connectorIds\":[\"LConn2\"],\"side\":\"TOP\"},\"type\":\"ConnectorPlacement.EquallySpacedRectSide\",\"uuid\":\"2a04a964-d53e-47ee-8c79-d53dd599bafe\"},{\"content\":{\"connectorIds\":[\"RConn2\"],\"side\":\"BOTTOM\"},\"type\":\"ConnectorPlacement.EquallySpacedRectSide\",\"uuid\":\"a0066dd6-a193-491c-afbe-bac00dfc3505\"}]},\"type\":\"ConnectorPlacement.EquallySpacedConnector\",\"uuid\":\"c80211c6-bb24-481b-97ca-2752015f3b18\"}],\"packageUris\":[\"http://schema.mathworks.com/mf0/Connector/19700101\"],\"version\":\"1.0\"}"
  Tile95 : Subsystem  mask(Square Tile){side=side, thickness=thick, color=color2, opacity=opacity}
      mask prompts: side "Side (m) :"; thickness "Thickness (m) :"; color "Color [RGB] :"; opacity "Opacity (0...1) :"
      mask help: This block creates a flat, single, square tile element. The square tile body is mass-less, so it will not have an effect on the dynamic simulation. This square tile element can be used as a graphic reference by itself, or as part of a composite graphic reference made of an array of interconnected tiles. The square tile is aligned with the XY plane, and the block provides frame connector ports to the middle points on each of the four sides of the body of the square - right (+X), left (-X), top (+Y) and bottom (-Y). All dimensions are in meters.
      settings: PortSchema="{\"entries\":[{\"content\":{\"sides\":[{\"content\":{\"connectorIds\":[\"LConn1\"]},\"type\":\"ConnectorPlacement.EquallySpacedRectSide\",\"uuid\":\"a971723f-ea37-4e9b-910b-501b94fb0ba2\"},{\"content\":{\"connectorIds\":[\"RConn1\"],\"side\":\"RIGHT\"},\"type\":\"ConnectorPlacement.EquallySpacedRectSide\",\"uuid\":\"e50175c1-005c-4b0b-bced-b882197eaab2\"},{\"content\":{\"connectorIds\":[\"LConn2\"],\"side\":\"TOP\"},\"type\":\"ConnectorPlacement.EquallySpacedRectSide\",\"uuid\":\"2a04a964-d53e-47ee-8c79-d53dd599bafe\"},{\"content\":{\"connectorIds\":[\"RConn2\"],\"side\":\"BOTTOM\"},\"type\":\"ConnectorPlacement.EquallySpacedRectSide\",\"uuid\":\"a0066dd6-a193-491c-afbe-bac00dfc3505\"}]},\"type\":\"ConnectorPlacement.EquallySpacedConnector\",\"uuid\":\"c80211c6-bb24-481b-97ca-2752015f3b18\"}],\"packageUris\":[\"http://schema.mathworks.com/mf0/Connector/19700101\"],\"version\":\"1.0\"}"
  Tile96 : Subsystem  mask(Square Tile){side=side, thickness=thick, color=color1, opacity=opacity}
      mask prompts: side "Side (m) :"; thickness "Thickness (m) :"; color "Color [RGB] :"; opacity "Opacity (0...1) :"
      mask help: This block creates a flat, single, square tile element. The square tile body is mass-less, so it will not have an effect on the dynamic simulation. This square tile element can be used as a graphic reference by itself, or as part of a composite graphic reference made of an array of interconnected tiles. The square tile is aligned with the XY plane, and the block provides frame connector ports to the middle points on each of the four sides of the body of the square - right (+X), left (-X), top (+Y) and bottom (-Y). All dimensions are in meters.
      settings: PortSchema="{\"entries\":[{\"content\":{\"sides\":[{\"content\":{\"connectorIds\":[\"LConn1\"]},\"type\":\"ConnectorPlacement.EquallySpacedRectSide\",\"uuid\":\"a971723f-ea37-4e9b-910b-501b94fb0ba2\"},{\"content\":{\"connectorIds\":[\"RConn1\"],\"side\":\"RIGHT\"},\"type\":\"ConnectorPlacement.EquallySpacedRectSide\",\"uuid\":\"e50175c1-005c-4b0b-bced-b882197eaab2\"},{\"content\":{\"connectorIds\":[\"LConn2\"],\"side\":\"TOP\"},\"type\":\"ConnectorPlacement.EquallySpacedRectSide\",\"uuid\":\"2a04a964-d53e-47ee-8c79-d53dd599bafe\"},{\"content\":{\"connectorIds\":[\"RConn2\"],\"side\":\"BOTTOM\"},\"type\":\"ConnectorPlacement.EquallySpacedRectSide\",\"uuid\":\"a0066dd6-a193-491c-afbe-bac00dfc3505\"}]},\"type\":\"ConnectorPlacement.EquallySpacedConnector\",\"uuid\":\"c80211c6-bb24-481b-97ca-2752015f3b18\"}],\"packageUris\":[\"http://schema.mathworks.com/mf0/Connector/19700101\"],\"version\":\"1.0\"}"
  Tile97 : Subsystem  mask(Square Tile){side=side, thickness=thick, color=color2, opacity=opacity}
      mask prompts: side "Side (m) :"; thickness "Thickness (m) :"; color "Color [RGB] :"; opacity "Opacity (0...1) :"
      mask help: This block creates a flat, single, square tile element. The square tile body is mass-less, so it will not have an effect on the dynamic simulation. This square tile element can be used as a graphic reference by itself, or as part of a composite graphic reference made of an array of interconnected tiles. The square tile is aligned with the XY plane, and the block provides frame connector ports to the middle points on each of the four sides of the body of the square - right (+X), left (-X), top (+Y) and bottom (-Y). All dimensions are in meters.
      settings: PortSchema="{\"entries\":[{\"content\":{\"sides\":[{\"content\":{\"connectorIds\":[\"LConn1\"]},\"type\":\"ConnectorPlacement.EquallySpacedRectSide\",\"uuid\":\"a971723f-ea37-4e9b-910b-501b94fb0ba2\"},{\"content\":{\"connectorIds\":[\"RConn1\"],\"side\":\"RIGHT\"},\"type\":\"ConnectorPlacement.EquallySpacedRectSide\",\"uuid\":\"e50175c1-005c-4b0b-bced-b882197eaab2\"},{\"content\":{\"connectorIds\":[\"LConn2\"],\"side\":\"TOP\"},\"type\":\"ConnectorPlacement.EquallySpacedRectSide\",\"uuid\":\"2a04a964-d53e-47ee-8c79-d53dd599bafe\"},{\"content\":{\"connectorIds\":[\"RConn2\"],\"side\":\"BOTTOM\"},\"type\":\"ConnectorPlacement.EquallySpacedRectSide\",\"uuid\":\"a0066dd6-a193-491c-afbe-bac00dfc3505\"}]},\"type\":\"ConnectorPlacement.EquallySpacedConnector\",\"uuid\":\"c80211c6-bb24-481b-97ca-2752015f3b18\"}],\"packageUris\":[\"http://schema.mathworks.com/mf0/Connector/19700101\"],\"version\":\"1.0\"}"
  Tile98 : Subsystem  mask(Square Tile){side=side, thickness=thick, color=color1, opacity=opacity}
      mask prompts: side "Side (m) :"; thickness "Thickness (m) :"; color "Color [RGB] :"; opacity "Opacity (0...1) :"
      mask help: This block creates a flat, single, square tile element. The square tile body is mass-less, so it will not have an effect on the dynamic simulation. This square tile element can be used as a graphic reference by itself, or as part of a composite graphic reference made of an array of interconnected tiles. The square tile is aligned with the XY plane, and the block provides frame connector ports to the middle points on each of the four sides of the body of the square - right (+X), left (-X), top (+Y) and bottom (-Y). All dimensions are in meters.
      settings: PortSchema="{\"entries\":[{\"content\":{\"sides\":[{\"content\":{\"connectorIds\":[\"LConn1\"]},\"type\":\"ConnectorPlacement.EquallySpacedRectSide\",\"uuid\":\"a971723f-ea37-4e9b-910b-501b94fb0ba2\"},{\"content\":{\"connectorIds\":[\"RConn1\"],\"side\":\"RIGHT\"},\"type\":\"ConnectorPlacement.EquallySpacedRectSide\",\"uuid\":\"e50175c1-005c-4b0b-bced-b882197eaab2\"},{\"content\":{\"connectorIds\":[\"LConn2\"],\"side\":\"TOP\"},\"type\":\"ConnectorPlacement.EquallySpacedRectSide\",\"uuid\":\"2a04a964-d53e-47ee-8c79-d53dd599bafe\"},{\"content\":{\"connectorIds\":[\"RConn2\"],\"side\":\"BOTTOM\"},\"type\":\"ConnectorPlacement.EquallySpacedRectSide\",\"uuid\":\"a0066dd6-a193-491c-afbe-bac00dfc3505\"}]},\"type\":\"ConnectorPlacement.EquallySpacedConnector\",\"uuid\":\"c80211c6-bb24-481b-97ca-2752015f3b18\"}],\"packageUris\":[\"http://schema.mathworks.com/mf0/Connector/19700101\"],\"version\":\"1.0\"}"
  Tile99 : Subsystem  mask(Square Tile){side=side, thickness=thick, color=color2, opacity=opacity}
      mask prompts: side "Side (m) :"; thickness "Thickness (m) :"; color "Color [RGB] :"; opacity "Opacity (0...1) :"
      mask help: This block creates a flat, single, square tile element. The square tile body is mass-less, so it will not have an effect on the dynamic simulation. This square tile element can be used as a graphic reference by itself, or as part of a composite graphic reference made of an array of interconnected tiles. The square tile is aligned with the XY plane, and the block provides frame connector ports to the middle points on each of the four sides of the body of the square - right (+X), left (-X), top (+Y) and bottom (-Y). All dimensions are in meters.
      settings: PortSchema="{\"entries\":[{\"content\":{\"sides\":[{\"content\":{\"connectorIds\":[\"LConn1\"]},\"type\":\"ConnectorPlacement.EquallySpacedRectSide\",\"uuid\":\"a971723f-ea37-4e9b-910b-501b94fb0ba2\"},{\"content\":{\"connectorIds\":[\"RConn1\"],\"side\":\"RIGHT\"},\"type\":\"ConnectorPlacement.EquallySpacedRectSide\",\"uuid\":\"e50175c1-005c-4b0b-bced-b882197eaab2\"},{\"content\":{\"connectorIds\":[\"LConn2\"],\"side\":\"TOP\"},\"type\":\"ConnectorPlacement.EquallySpacedRectSide\",\"uuid\":\"2a04a964-d53e-47ee-8c79-d53dd599bafe\"},{\"content\":{\"connectorIds\":[\"RConn2\"],\"side\":\"BOTTOM\"},\"type\":\"ConnectorPlacement.EquallySpacedRectSide\",\"uuid\":\"a0066dd6-a193-491c-afbe-bac00dfc3505\"}]},\"type\":\"ConnectorPlacement.EquallySpacedConnector\",\"uuid\":\"c80211c6-bb24-481b-97ca-2752015f3b18\"}],\"packageUris\":[\"http://schema.mathworks.com/mf0/Connector/19700101\"],\"version\":\"1.0\"}"
  F : PMIOPort  Side=Left
  connections:
  F/RConn1 -- Tile1/LConn1
  Tile2/LConn1 -- Tile1/RConn1
  Tile4/LConn1 -- Tile3/RConn1
  Tile2/RConn1 -- Tile3/LConn1
  Tile6/RConn1 -- Tile7/LConn1
  Tile8/LConn1 -- Tile7/RConn1
  Tile6/LConn1 -- Tile5/RConn1
  Tile5/LConn1 -- Tile4/RConn1
  Tile10/LConn1 -- Tile9/RConn1
  Tile9/LConn1 -- Tile8/RConn1
  Tile15/LConn1 -- Tile14/RConn1
  Tile16/LConn1 -- Tile15/RConn1
  Tile16/RConn1 -- Tile17/LConn1
  Tile18/LConn1 -- Tile17/RConn1
  Tile11/LConn1 -- Tile19/RConn1
  Tile19/LConn1 -- Tile18/RConn1
  Tile12/RConn1 -- Tile13/LConn1
  Tile14/LConn1 -- Tile13/RConn1
  Tile12/LConn2 -- Tile1/RConn2
  Tile20/LConn1 -- Tile11/RConn1
  Tile24/LConn2 -- Tile21/RConn2
  Tile26/LConn1 -- Tile25/RConn1
  Tile24/RConn1 -- Tile25/LConn1
  Tile31/LConn1 -- Tile30/RConn1
  Tile30/LConn1 -- Tile29/RConn1
  Tile23/LConn1 -- Tile31/RConn1
  Tile28/RConn1 -- Tile29/LConn1
  Tile28/LConn1 -- Tile27/RConn1
  Tile27/LConn1 -- Tile26/RConn1
  Tile36/LConn1 -- Tile35/RConn1
  Tile37/LConn1 -- Tile36/RConn1
  Tile22/LConn1 -- Tile40/RConn1
  Tile37/RConn1 -- Tile38/LConn1
  Tile40/LConn1 -- Tile39/RConn1
  Tile39/LConn1 -- Tile38/RConn1
  Tile32/RConn1 -- Tile34/LConn1
  Tile35/LConn1 -- Tile34/RConn1
  Tile32/LConn1 -- Tile21/RConn1
  Tile33/LConn1 -- Tile23/RConn1
  Tile21/LConn2 -- Tile12/RConn2
  Tile43/LConn1 -- Tile41/RConn1
  Tile43/RConn1 -- Tile44/LConn1
  Tile49/LConn1 -- Tile48/RConn1
  Tile50/LConn1 -- Tile49/RConn1
  Tile42/LConn1 -- Tile50/RConn1
  Tile47/RConn1 -- Tile48/LConn1
  Tile47/LConn1 -- Tile46/RConn1
  Tile46/LConn1 -- Tile45/RConn1
  Tile45/LConn1 -- Tile44/RConn1
  Tile41/LConn2 -- Tile24/RConn2
  Tile55/LConn1 -- Tile54/RConn1
  Tile56/LConn1 -- Tile55/RConn1
  Tile56/RConn1 -- Tile57/LConn1
  Tile58/LConn1 -- Tile57/RConn1
  Tile52/RConn1 -- Tile53/LConn1
  Tile51/LConn1 -- Tile59/RConn1
  Tile60/LConn1 -- Tile51/RConn1
  Tile54/LConn1 -- Tile53/RConn1
  Tile59/LConn1 -- Tile58/RConn1
  Tile52/LConn2 -- Tile41/RConn2
  Tile109/LConn1 -- Tile108/RConn1
  Tile110/LConn1 -- Tile101/RConn1
  Tile91/LConn2 -- Tile74/RConn2
  Tile95/LConn1 -- Tile94/RConn1
  Tile97/RConn1 -- Tile98/LConn1
  Tile108/LConn1 -- Tile107/RConn1
  Tile100/LConn1 -- Tile99/RConn1
  Tile99/LConn1 -- Tile98/RConn1
  Tile93/RConn1 -- Tile94/LConn1
  Tile85/LConn1 -- Tile84/RConn1
  Tile89/LConn1 -- Tile88/RConn1
  Tile93/LConn1 -- Tile91/RConn1
  Tile90/LConn1 -- Tile89/RConn1
  Tile87/RConn1 -- Tile88/LConn1
  Tile72/LConn1 -- Tile90/RConn1
  Tile96/LConn1 -- Tile95/RConn1
  Tile87/LConn1 -- Tile86/RConn1
  Tile105/LConn1 -- Tile104/RConn1
  Tile86/LConn1 -- Tile85/RConn1
  Tile77/LConn1 -- Tile76/RConn1
  Tile78/LConn1 -- Tile77/RConn1
  Tile82/RConn1 -- Tile84/LConn1
  Tile78/RConn1 -- Tile79/LConn1
  Tile73/LConn1 -- Tile81/RConn1
  Tile80/LConn1 -- Tile79/RConn1
  Tile81/LConn1 -- Tile80/RConn1
  Tile76/LConn1 -- Tile75/RConn1
  Tile74/LConn2 -- Tile71/RConn2
  Tile92/LConn1 -- Tile100/RConn1
  Tile104/LConn1 -- Tile103/RConn1
  Tile102/LConn2 -- Tile91/RConn2
  Tile83/LConn1 -- Tile73/RConn1
  Tile106/RConn1 -- Tile107/LConn1
  Tile74/RConn1 -- Tile75/LConn1
  Tile97/LConn1 -- Tile96/RConn1
  Tile106/LConn1 -- Tile105/RConn1
  Tile101/LConn1 -- Tile109/RConn1
  Tile82/LConn1 -- Tile71/RConn1
  Tile102/RConn1 -- Tile103/LConn1
  Tile1/LConn2 -- Tile102/RConn2
  Tile70/LConn1 -- Tile61/RConn1
  Tile69/LConn1 -- Tile68/RConn1
  Tile62/RConn1 -- Tile63/LConn1
  Tile61/LConn1 -- Tile69/RConn1
  Tile66/RConn1 -- Tile67/LConn1
  Tile68/LConn1 -- Tile67/RConn1
  Tile65/LConn1 -- Tile64/RConn1
  Tile66/LConn1 -- Tile65/RConn1
  Tile64/LConn1 -- Tile63/RConn1
  Tile62/RConn2 -- Tile71/LConn2
  Tile70/RConn1 -- Tile118/LConn1
  Tile72/RConn1 -- Tile121/LConn1
  Tile83/RConn1 -- Tile119/LConn1
  Tile92/RConn1 -- Tile111/LConn1
  Tile110/RConn1 -- Tile112/LConn1
  Tile10/RConn1 -- Tile120/LConn1
  Tile20/RConn1 -- Tile113/LConn1
  Tile22/RConn1 -- Tile115/LConn1
  Tile33/RConn1 -- Tile114/LConn1
  Tile42/RConn1 -- Tile116/LConn1
  Tile60/RConn1 -- Tile117/LConn1
  Tile152/RConn1 -- Tile134/LConn1
  Tile147/RConn1 -- Tile133/LConn1
  Tile141/RConn1 -- Tile132/LConn1
  Tile140/RConn1 -- Tile130/LConn1
  Tile122/RConn1 -- Tile137/LConn1
  Tile144/RConn1 -- Tile131/LConn1
  Tile127/RConn1 -- Tile129/LConn1
  Tile160/RConn1 -- Tile136/LConn1
  Tile156/RConn1 -- Tile138/LConn1
  Tile153/LConn1 -- Tile154/RConn1
  Tile124/LConn1 -- Tile125/RConn1
  Tile160/LConn1 -- Tile157/RConn1
  Tile157/LConn1 -- Tile159/RConn1
  Tile164/LConn1 -- Tile123/RConn1
  Tile156/LConn1 -- Tile163/RConn1
  Tile163/LConn1 -- Tile161/RConn1
  Tile127/LConn1 -- Tile124/RConn1
  Tile155/LConn1 -- Tile153/RConn1
  Tile152/LConn1 -- Tile150/RConn1
  Tile147/LConn1 -- Tile149/RConn1
  Tile141/LConn1 -- Tile146/RConn1
  Tile150/LConn1 -- Tile151/RConn1
  Tile142/LConn1 -- Tile143/RConn1
  Tile146/LConn1 -- Tile145/RConn1
  Tile140/LConn1 -- Tile126/RConn1
  Tile162/LConn1 -- Tile158/RConn1
  Tile126/LConn1 -- Tile139/RConn1
  Tile164/RConn1 -- Tile128/LConn1
  Tile144/LConn1 -- Tile142/RConn1
  Tile123/LConn1 -- Tile165/RConn1
  Tile122/LConn1 -- Tile162/RConn1
  Tile149/LConn1 -- Tile148/RConn1
  Tile155/RConn1 -- Tile135/LConn1
  Tile118/RConn1 -- Tile154/LConn1
  Tile121/RConn1 -- Tile161/LConn1
  Tile119/RConn1 -- Tile159/LConn1
  Tile111/RConn1 -- Tile165/LConn1
  Tile112/RConn1 -- Tile125/LConn1
  Tile120/RConn1 -- Tile158/LConn1
  Tile113/RConn1 -- Tile139/LConn1
  Tile115/RConn1 -- Tile145/LConn1
  Tile114/RConn1 -- Tile143/LConn1
  Tile116/RConn1 -- Tile148/LConn1
  Tile117/RConn1 -- Tile151/LConn1
  Tile167/RConn1 -- Tile174/LConn1
  Tile166/RConn1 -- Tile171/LConn1
  Tile172/LConn1 -- Tile171/RConn1
  Tile173/LConn1 -- Tile174/RConn1
  Tile170/LConn1 -- Tile172/RConn1
  Tile175/LConn1 -- Tile173/RConn1
  Tile170/RConn1 -- Tile168/LConn1
  Tile195/RConn1 -- Tile167/LConn1
  Tile177/RConn1 -- Tile166/LConn1
  Tile187/LConn2 -- Tile176/RConn2
  Tile194/LConn1 -- Tile193/RConn1
  Tile189/LConn1 -- Tile188/RConn1
  Tile195/LConn1 -- Tile186/RConn1
  Tile186/LConn1 -- Tile194/RConn1
  Tile193/LConn1 -- Tile192/RConn1
  Tile187/RConn1 -- Tile188/LConn1
  Tile175/RConn1 -- Tile169/LConn1
  Tile191/RConn1 -- Tile192/LConn1
  Tile191/LConn1 -- Tile190/RConn1
  Tile190/LConn1 -- Tile189/RConn1
  Tile52/RConn2 -- Tile176/LConn2
  Tile177/LConn1 -- Tile185/RConn1
  Tile182/RConn1 -- Tile183/LConn1
  Tile180/LConn1 -- Tile179/RConn1
  Tile181/LConn1 -- Tile180/RConn1
  Tile185/LConn1 -- Tile184/RConn1
  Tile184/LConn1 -- Tile183/RConn1
  Tile182/LConn1 -- Tile181/RConn1
  Tile178/RConn1 -- Tile179/LConn1
  Tile178/LConn1 -- Tile176/RConn1
  Tile196/RConn1 -- Tile201/LConn1
  Tile202/RConn1 -- Tile198/LConn1
  Tile202/LConn1 -- Tile200/RConn1
  Tile217/RConn1 -- Tile197/LConn1
  Tile215/RConn1 -- Tile196/LConn1
  Tile207/RConn2 -- Tile216/LConn2
  Tile209/LConn1 -- Tile208/RConn1
  Tile211/LConn1 -- Tile210/RConn1
  Tile210/LConn1 -- Tile209/RConn1
  Tile205/LConn1 -- Tile204/RConn1
  Tile213/LConn1 -- Tile212/RConn1
  Tile211/RConn1 -- Tile212/LConn1
  Tile203/LConn1 -- Tile205/RConn1
  Tile206/LConn1 -- Tile214/RConn1
  Tile207/RConn1 -- Tile208/LConn1
  Tile214/LConn1 -- Tile213/RConn1
  Tile200/LConn1 -- Tile201/RConn1
  Tile215/LConn1 -- Tile206/RConn1
  Tile218/RConn1 -- Tile219/LConn1
  Tile222/LConn1 -- Tile221/RConn1
  Tile217/LConn1 -- Tile225/RConn1
  Tile225/LConn1 -- Tile224/RConn1
  Tile222/RConn1 -- Tile223/LConn1
  Tile221/LConn1 -- Tile220/RConn1
  Tile218/LConn1 -- Tile216/RConn1
  Tile224/LConn1 -- Tile223/RConn1
  Tile197/RConn1 -- Tile204/LConn1
  Tile220/LConn1 -- Tile219/RConn1
  Tile203/RConn1 -- Tile199/LConn1
  Tile216/RConn2 -- Tile62/LConn2
  Tile245/LConn1 -- Tile244/RConn1
  Tile260/LConn1 -- Tile259/RConn1
  Tile258/LConn1 -- Tile256/RConn1
  Tile256/RConn2 -- Tile267/LConn2
  Tile254/LConn1 -- Tile253/RConn1
  Tile236/RConn1 -- Tile241/LConn1
  Tile275/RConn1 -- Tile226/LConn1
  Tile233/LConn1 -- Tile235/RConn1
  Tile255/RConn1 -- Tile236/LConn1
  Tile282/RConn1 -- Tile283/LConn1
  Tile237/RConn1 -- Tile244/LConn1
  Tile267/RConn2 -- Tile276/LConn2
  Tile270/LConn1 -- Tile269/RConn1
  Tile262/LConn1 -- Tile261/RConn1
  Tile253/LConn1 -- Tile252/RConn1
  Tile264/LConn1 -- Tile263/RConn1
  Tile251/RConn1 -- Tile252/LConn1
  Tile282/LConn1 -- Tile281/RConn1
  Tile232/RConn1 -- Tile228/LConn1
  Tile258/RConn1 -- Tile259/LConn1
  Tile265/LConn1 -- Tile264/RConn1
  Tile247/RConn2 -- Tile256/LConn2
  Tile246/LConn1 -- Tile254/RConn1
  Tile284/LConn1 -- Tile283/RConn1
  Tile274/LConn1 -- Tile273/RConn1
  Tile227/RConn1 -- Tile234/LConn1
  Tile271/RConn1 -- Tile272/LConn1
  Tile255/LConn1 -- Tile246/RConn1
  Tile247/RConn1 -- Tile248/LConn1
  Tile226/RConn1 -- Tile231/LConn1
  Tile266/LConn1 -- Tile274/RConn1
  Tile207/LConn2 -- Tile276/RConn2
  Tile275/LConn1 -- Tile266/RConn1
  Tile250/LConn1 -- Tile249/RConn1
  Tile233/RConn1 -- Tile229/LConn1
  Tile280/LConn1 -- Tile279/RConn1
  Tile267/RConn1 -- Tile268/LConn1
  Tile261/LConn1 -- Tile260/RConn1
  Tile273/LConn1 -- Tile272/RConn1
  Tile249/LConn1 -- Tile248/RConn1
  Tile242/LConn1 -- Tile240/RConn1
  Tile251/LConn1 -- Tile250/RConn1
  Tile242/RConn1 -- Tile238/LConn1
  Tile257/LConn1 -- Tile265/RConn1
  Tile257/RConn1 -- Tile237/LConn1
  Tile285/LConn1 -- Tile284/RConn1
  Tile269/LConn1 -- Tile268/RConn1
  Tile277/LConn1 -- Tile285/RConn1
  Tile271/LConn1 -- Tile270/RConn1
  Tile277/RConn1 -- Tile227/LConn1
  Tile243/LConn1 -- Tile245/RConn1
  Tile230/LConn1 -- Tile231/RConn1
  Tile278/RConn1 -- Tile279/LConn1
  Tile278/LConn1 -- Tile276/RConn1
  Tile235/LConn1 -- Tile234/RConn1
  Tile262/RConn1 -- Tile263/LConn1
  Tile281/LConn1 -- Tile280/RConn1
  Tile232/LConn1 -- Tile230/RConn1
  Tile240/LConn1 -- Tile241/RConn1
  Tile243/RConn1 -- Tile239/LConn1
  Tile308/LConn1 -- Tile306/RConn1
  Tile308/RConn1 -- Tile309/LConn1
  Tile312/LConn1 -- Tile311/RConn1
  Tile314/LConn1 -- Tile313/RConn1
  Tile315/LConn1 -- Tile314/RConn1
  Tile310/LConn1 -- Tile309/RConn1
  Tile312/RConn1 -- Tile313/LConn1
  Tile307/LConn1 -- Tile315/RConn1
  Tile305/RConn1 -- Tile299/LConn1
  Tile317/RConn1 -- Tile318/LConn1
  Tile319/LConn1 -- Tile318/RConn1
  Tile317/LConn2 -- Tile306/RConn2
  Tile307/RConn1 -- Tile296/LConn1
  Tile323/LConn1 -- Tile322/RConn1
  Tile311/LConn1 -- Tile310/RConn1
  Tile325/RConn1 -- Tile297/LConn1
  Tile300/RConn1 -- Tile298/LConn1
  Tile305/LConn1 -- Tile303/RConn1
  Tile300/LConn1 -- Tile302/RConn1
  Tile303/LConn1 -- Tile304/RConn1
  Tile296/RConn1 -- Tile301/LConn1
  Tile286/RConn1 -- Tile291/LConn1
  Tile321/RConn1 -- Tile322/LConn1
  Tile292/LConn1 -- Tile291/RConn1
  Tile297/RConn1 -- Tile304/LConn1
  Tile295/LConn1 -- Tile293/RConn1
  Tile295/RConn1 -- Tile289/LConn1
  Tile287/RConn1 -- Tile294/LConn1
  Tile345/RConn1 -- Tile287/LConn1
  Tile293/LConn1 -- Tile294/RConn1
  Tile327/RConn1 -- Tile286/LConn1
  Tile337/RConn2 -- Tile306/LConn2
  Tile337/LConn2 -- Tile326/RConn2
  Tile344/LConn1 -- Tile343/RConn1
  Tile339/LConn1 -- Tile338/RConn1
  Tile321/LConn1 -- Tile320/RConn1
  Tile336/LConn1 -- Tile344/RConn1
  Tile337/RConn1 -- Tile338/LConn1
  Tile290/LConn1 -- Tile292/RConn1
  Tile320/LConn1 -- Tile319/RConn1
  Tile343/LConn1 -- Tile342/RConn1
  Tile341/RConn1 -- Tile342/LConn1
  Tile302/LConn1 -- Tile301/RConn1
  Tile341/LConn1 -- Tile340/RConn1
  Tile340/LConn1 -- Tile339/RConn1
  Tile187/RConn2 -- Tile326/LConn2
  Tile331/LConn1 -- Tile330/RConn1
  Tile316/LConn1 -- Tile324/RConn1
  Tile332/LConn1 -- Tile331/RConn1
  Tile290/RConn1 -- Tile288/LConn1
  Tile330/LConn1 -- Tile329/RConn1
  Tile327/LConn1 -- Tile335/RConn1
  Tile324/LConn1 -- Tile323/RConn1
  Tile335/LConn1 -- Tile334/RConn1
  Tile325/LConn1 -- Tile316/RConn1
  Tile334/LConn1 -- Tile333/RConn1
  Tile328/LConn1 -- Tile326/RConn1
  Tile345/LConn1 -- Tile336/RConn1
  Tile328/RConn1 -- Tile329/LConn1
  Tile332/RConn1 -- Tile333/LConn1
  Tile508/LConn1 -- Tile506/RConn1
  Tile288/RConn1 -- Tile504/LConn1
  Tile501/LConn1 -- Tile499/RConn1
  Tile505/LConn1 -- Tile504/RConn1
  Tile299/RConn1 -- Tile500/LConn1
  Tile502/LConn1 -- Tile505/RConn1
  Tile479/RConn1 -- Tile477/LConn1
  Tile499/LConn1 -- Tile500/RConn1
  Tile479/LConn1 -- Tile481/RConn1
  Tile502/RConn1 -- Tile475/LConn1
  Tile482/LConn1 -- Tile483/RConn1
  Tile508/RConn1 -- Tile476/LConn1
  Tile484/RConn1 -- Tile478/LConn1
  Tile486/RConn1 -- Tile493/LConn1
  Tile481/LConn1 -- Tile480/RConn1
  Tile289/RConn1 -- Tile507/LConn1
  Tile475/RConn1 -- Tile480/LConn1
  Tile492/LConn1 -- Tile493/RConn1
  Tile489/LConn1 -- Tile491/RConn1
  Tile494/LConn1 -- Tile492/RConn1
  Tile489/RConn1 -- Tile487/LConn1
  Tile501/RConn1 -- Tile486/LConn1
  Tile495/RConn1 -- Tile485/LConn1
  Tile494/RConn1 -- Tile488/LConn1
  Tile498/LConn1 -- Tile497/RConn1
  Tile460/RConn1 -- Tile456/LConn1
  Tile457/LConn1 -- Tile458/RConn1
  Tile447/LConn1 -- Tile448/RConn1
  Tile460/LConn1 -- Tile462/RConn1
  Tile472/LConn1 -- Tile474/RConn1
  Tile466/RConn1 -- Tile454/LConn1
  Tile472/RConn1 -- Tile443/LConn1
  Tile466/LConn1 -- Tile468/RConn1
  Tile459/LConn1 -- Tile457/RConn1
  Tile450/RConn1 -- Tile445/LConn1
  Tile469/LConn1 -- Tile470/RConn1
  Tile442/RConn1 -- Tile448/LConn1
  Tile465/LConn1 -- Tile463/RConn1
  Tile443/RConn1 -- Tile451/LConn1
  Tile228/RConn1 -- Tile470/LConn1
  Tile229/RConn1 -- Tile473/LConn1
  Tile463/LConn1 -- Tile464/RConn1
  Tile468/LConn1 -- Tile467/RConn1
  Tile449/RConn1 -- Tile444/LConn1
  Tile239/RConn1 -- Tile467/LConn1
  Tile454/RConn1 -- Tile461/LConn1
  Tile465/RConn1 -- Tile453/LConn1
  Tile471/RConn1 -- Tile442/LConn1
  Tile453/RConn1 -- Tile458/LConn1
  Tile462/LConn1 -- Tile461/RConn1
  Tile425/RConn1 -- Tile433/LConn1
  Tile441/LConn1 -- Tile440/RConn1
  Tile474/LConn1 -- Tile473/RConn1
  Tile438/LConn1 -- Tile441/RConn1
  Tile437/LConn1 -- Tile435/RConn1
  Tile429/LConn1 -- Tile430/RConn1
  Tile198/RConn1 -- Tile436/LConn1
  Tile435/LConn1 -- Tile436/RConn1
  Tile452/LConn1 -- Tile451/RConn1
  Tile432/LConn1 -- Tile434/RConn1
  Tile434/LConn1 -- Tile433/RConn1
  Tile437/RConn1 -- Tile424/LConn1
  Tile438/RConn1 -- Tile425/LConn1
  Tile431/LConn1 -- Tile429/RConn1
  Tile424/RConn1 -- Tile430/LConn1
  Tile168/RConn1 -- Tile418/LConn1
  Tile419/LConn1 -- Tile418/RConn1
  Tile417/LConn1 -- Tile419/RConn1
  Tile416/RConn1 -- Tile410/LConn1
  Tile420/LConn1 -- Tile422/RConn1
  Tile423/LConn1 -- Tile420/RConn1
  Tile169/RConn1 -- Tile422/LConn1
  Tile476/RConn1 -- Tile483/LConn1
  Tile417/RConn1 -- Tile407/LConn1
  Tile423/RConn1 -- Tile408/LConn1
  Tile411/RConn1 -- Tile409/LConn1
  Tile484/LConn1 -- Tile482/RConn1
  Tile416/LConn1 -- Tile414/RConn1
  Tile411/LConn1 -- Tile413/RConn1
  Tile414/LConn1 -- Tile415/RConn1
  Tile450/LConn1 -- Tile452/RConn1
  Tile413/LConn1 -- Tile412/RConn1
  Tile407/RConn1 -- Tile412/LConn1
  Tile459/RConn1 -- Tile455/LConn1
  Tile408/RConn1 -- Tile415/LConn1
  Tile357/RConn1 -- Tile389/LConn1
  Tile355/RConn1 -- Tile384/LConn1
  Tile356/RConn1 -- Tile386/LConn1
  Tile354/RConn1 -- Tile380/LConn1
  Tile491/LConn1 -- Tile490/RConn1
  Tile361/RConn1 -- Tile399/LConn1
  Tile353/RConn1 -- Tile366/LConn1
  Tile352/RConn1 -- Tile406/LConn1
  Tile360/RConn1 -- Tile400/LConn1
  Tile362/RConn1 -- Tile402/LConn1
  Tile359/RConn1 -- Tile395/LConn1
  Tile396/RConn1 -- Tile376/LConn1
  Tile298/RConn1 -- Tile497/LConn1
  Tile363/LConn1 -- Tile403/RConn1
  Tile431/RConn1 -- Tile426/LConn1
  Tile364/LConn1 -- Tile406/RConn1
  Tile385/LConn1 -- Tile383/RConn1
  Tile405/RConn1 -- Tile369/LConn1
  Tile403/LConn1 -- Tile399/RConn1
  Tile381/LConn1 -- Tile367/RConn1
  Tile387/LConn1 -- Tile386/RConn1
  Tile390/LConn1 -- Tile389/RConn1
  Tile383/LConn1 -- Tile384/RConn1
  Tile388/LConn1 -- Tile390/RConn1
  Tile393/LConn1 -- Tile391/RConn1
  Tile396/LConn1 -- Tile394/RConn1
  Tile368/LConn1 -- Tile365/RConn1
  Tile495/LConn1 -- Tile498/RConn1
  Tile397/LConn1 -- Tile404/RConn1
  Tile432/RConn1 -- Tile427/LConn1
  Tile405/LConn1 -- Tile364/RConn1
  Tile398/LConn1 -- Tile400/RConn1
  Tile365/LConn1 -- Tile366/RConn1
  Tile199/RConn1 -- Tile440/LConn1
  Tile394/LConn1 -- Tile395/RConn1
  Tile401/RConn1 -- Tile377/LConn1
  Tile368/RConn1 -- Tile370/LConn1
  Tile363/RConn1 -- Tile378/LConn1
  Tile381/RConn1 -- Tile371/LConn1
  Tile397/RConn1 -- Tile379/LConn1
  Tile382/RConn1 -- Tile373/LConn1
  Tile388/RConn1 -- Tile374/LConn1
  Tile516/RConn1 -- Tile358/LConn1
  Tile391/LConn1 -- Tile392/RConn1
  Tile511/RConn1 -- Tile357/LConn1
  Tile382/LConn1 -- Tile387/RConn1
  Tile428/RConn1 -- Tile354/LConn1
  Tile367/LConn1 -- Tile380/RConn1
  Tile528/RConn1 -- Tile352/LConn1
  Tile346/RConn1 -- Tile361/LConn1
  Tile524/RConn1 -- Tile360/LConn1
  Tile503/RConn1 -- Tile355/LConn1
  Tile520/RConn1 -- Tile362/LConn1
  Tile401/LConn1 -- Tile398/RConn1
  Tile519/LConn1 -- Tile517/RConn1
  Tile517/LConn1 -- Tile518/RConn1
  Tile506/LConn1 -- Tile507/RConn1
  Tile348/LConn1 -- Tile349/RConn1
  Tile524/LConn1 -- Tile521/RConn1
  Tile358/RConn1 -- Tile392/LConn1
  Tile485/RConn1 -- Tile490/LConn1
  Tile393/RConn1 -- Tile375/LConn1
  Tile351/RConn1 -- Tile353/LConn1
  Tile528/LConn1 -- Tile347/RConn1
  Tile520/LConn1 -- Tile527/RConn1
  Tile471/LConn1 -- Tile469/RConn1
  Tile138/RConn1 -- Tile525/LConn1
  Tile128/RConn1 -- Tile529/LConn1
  Tile136/RConn1 -- Tile523/LConn1
  Tile347/LConn1 -- Tile529/RConn1
  Tile527/LConn1 -- Tile525/RConn1
  Tile129/RConn1 -- Tile349/LConn1
  Tile404/LConn1 -- Tile402/RConn1
  Tile134/RConn1 -- Tile515/LConn1
  Tile516/LConn1 -- Tile514/RConn1
  Tile514/LConn1 -- Tile515/RConn1
  Tile511/LConn1 -- Tile513/RConn1
  Tile351/LConn1 -- Tile348/RConn1
  Tile133/RConn1 -- Tile512/LConn1
  Tile385/RConn1 -- Tile372/LConn1
  Tile503/LConn1 -- Tile446/RConn1
  Tile132/RConn1 -- Tile509/LConn1
  Tile135/RConn1 -- Tile518/LConn1
  Tile513/LConn1 -- Tile512/RConn1
  Tile510/LConn1 -- Tile509/RConn1
  Tile439/LConn1 -- Tile510/RConn1
  Tile519/RConn1 -- Tile359/LConn1
  Tile131/RConn1 -- Tile496/LConn1
  Tile238/RConn1 -- Tile464/LConn1
  Tile350/LConn1 -- Tile421/RConn1
  Tile428/LConn1 -- Tile350/RConn1
  Tile526/LConn1 -- Tile522/RConn1
  Tile446/LConn1 -- Tile496/RConn1
  Tile449/LConn1 -- Tile447/RConn1
  Tile130/RConn1 -- Tile421/LConn1
  Tile439/RConn1 -- Tile356/LConn1
  Tile346/LConn1 -- Tile526/RConn1
  Tile137/RConn1 -- Tile522/LConn1
  Tile521/LConn1 -- Tile523/RConn1
